simulink model "motor"  (Simulink 8.6)
settings: Solver=FixedStepDiscrete  StartTime=0.0  StopTime=inf  FixedStep=0.002  RelTol=1e-3
PostLoadFcn:
  | ,try, rti_mdl_postloadfcn(bdroot, 'UpdateModel', 160, 'rti1104'); catch, disp(lasterr); end,
undefined symbols (not defined in the file): DiscIntNeverNeededParam
(part 3 of 3)

== stateflow chart Chart ==
  state Ready
    en:
    Cur_Limit=2200;%电流报警阈值
    Cur_GZ_Limit=2450;%电流故障阈值
    Temp_Up_Limit=2130;%温度上限阈值80°C
    Temp_Down_Limit=80;%温度下限阈值-45°C
    Open_Result=2;%开机结果失败
    Ini_Result=0;%初始化结果失败
    QDQ_BJ=1;%默认驱动器正常，1正常，2报警，3故障
    In_State=0;%状态标识，1表示初始化状态，2开机状态，3关机状态
    QDQ_XH=0;%QDQ_XH引脚状态，低
    QDQ_HY=1;%QDQ_HY引脚状态，高
    Motor_En=1;%电机使能引脚置高
    DCZD=1;%电磁制动引脚拉高，关电制动，低有效
    KG_clc=0;
    Alarm_Cunt=1;%实现程序中主动上报只执行发送一次
    Flag_Up_limit=1;%上限位标识，1正常，0报警
    Flag_Down_limit=1;%下限位标识，1正常，0报警
    Flag_Cur=1;%电流报警
    Flag_Temp_Up=1;%温度过高标识
    Flag_GXDY_Error=1;%惯性单元数据异常标识
    Flag_Enc_Error=1;%编码器标识，1正常，0故障
    Flag_Motor_Error=1;%电机正反转标识，1正常，0故障
    Flag_GZ_Cur=1;%电流过高故障
    Flag_Down_GZ_limit= 1;%下限位开关故障标识，1正常，0故障
    Flag_Up_GZ_limit= 1;%上限位开关故障标识，1正常，0故障
    Flag_Temp_Down=1;%温度过低标识，1正常，0故障
    Flag_GXDY_IT=1;%惯性单元通讯中断标识
    PWM_Value_Up= uint16(3300);%电机初始化上行PWM值
    PWM_Value_Down= uint16(1700);%电机初始化下行PWM值
    PWM_Value_Mid= uint16(2500);%PWM中指
    Encode_Sp_Max=3000;%换算编码器测速最大值
    Encode_Sp_Min= uint32(2);%编码器测速最小值
    Encode_Pos1=int32(-1161718);%下滑纵摇XHZY下机械限位位置
    Encode_Pos2=int32(-1155272);%下滑横摇XHHY下机械限位位置
    Encode_Pos3=int32(-1163716);%横摇灯杆XYDG下机械限位位置
    Encode_Pos_Zero=1000;%零点检测，回到零点时的范围
    Encode_Pos_Min=uint32(1400);%最小行程，检测电机是否正常运转
    JD_Max=uint32(20000);%角度变化最大值,
    Ts=double(0.002);%采样时间
  state Ready_Run
    state Current_check [parallel]
      settings: executionOrder=1
      state p1
        entry: cur_i=uint16(0);%计数器置零
        Flag_Cur=uint8(1);%电流正常
      state p4
        en:cur_i= uint16(1);
        du:cur_i = cur_i + 1;
      state p3
        %0代表正常，1代表错误
        entry: cur_i= uint16(0);
        Flag_Cur=uint8(0);%电流过流
        Flag_GZ_Cur=1;%电流未故障
      state p2
        en:cur_i=uint16(1);
        du:cur_i = cur_i + 1;
      state p5
        en:cur_i=uint16(1);
        du:cur_i = cur_i + 1;
      state p7
        en:cur_i= uint16(1);
        du:cur_i = cur_i + 1;
      state p6
        entry:%Motor_En=1;%电机失能
        Flag_GZ_Cur=uint8(0);%电流过流
      (default) -> Ready_Run.Current_check.p1
      Ready_Run.Current_check.p4 -> Ready_Run.Current_check.p1 [order 2] : [cur_i>=uint16(2/Ts)]
      Ready_Run.Current_check.p1 -> Ready_Run.Current_check.p2 : [Cur_In>=Cur_Limit]
      Ready_Run.Current_check.p2 -> Ready_Run.Current_check.p1 [order 1] : [Cur_In<Cur_Limit]
      Ready_Run.Current_check.p4 -> Ready_Run.Current_check.p3 [order 1] : [Cur_In>=Cur_Limit]
      Ready_Run.Current_check.p3 -> Ready_Run.Current_check.p4 [order 1] : [Cur_In<Cur_Limit]
      Ready_Run.Current_check.p7 -> Ready_Run.Current_check.p3 [order 2] : [cur_i>=uint16(2/Ts)]
      Ready_Run.Current_check.p2 -> Ready_Run.Current_check.p3 [order 2] : [cur_i>=uint16(2/Ts)]%2S
      Ready_Run.Current_check.p3 -> Ready_Run.Current_check.p5 [order 2] : [Cur_In>=Cur_GZ_Limit]
      Ready_Run.Current_check.p5 -> Ready_Run.Current_check.p3 [order 2] : [Cur_In<Cur_GZ_Limit]
      Ready_Run.Current_check.p5 -> Ready_Run.Current_check.p6 [order 1] : [cur_i>=uint16(2/Ts)]%2S
      Ready_Run.Current_check.p6 -> Ready_Run.Current_check.p7 : [Cur_In<Cur_GZ_Limit]
      Ready_Run.Current_check.p7 -> Ready_Run.Current_check.p6 [order 1] : [Cur_In>=Cur_GZ_Limit]
    state M_Run [parallel]
      entry:Encode_Pos0=Encode_Sp+Encode_Pos0;
      during:Encode_Pos0=Encode_Sp+Encode_Pos0;
      Encode_Pos=Encode_Pos0-Encode_Pos_Zero_Average;
      settings: executionOrder=3
      state Initialize
        entry:Ini_Result=uint8(0);%初始化失败
        In_State=1;
        state Parameters_Reset
          entry:
          Motor_En=0;%开电机
          Encode_Pos0= int32(0);%位置初始值
          chu_jd=0;
          KG=1;
        state hy
          state P5
            en:PWMOUT=PWM_Value_Up;
            du:PWMOUT=PWM_Value_Up;%电机上行
            on after(4/Ts,tick):Flag_Down_GZ_limit=0;%下限位开关故障
            %Motor_En=1;
            %PWMOUT=PWM_Value_Mid;
            %4S之后停机
          state P3
            en:PWMOUT=PWM_Value_Down;
            du:PWMOUT=PWM_Value_Down;%电机下行*/
            on after(4/Ts,tick):Flag_Up_GZ_limit= uint8(0);%上限位开关故障*/
            %Motor_En=1;
            %电机失能，关
            %PWMOUT=PWM_Value_Mid;
            %4S之后停机*/
          state P4
            en:chu_jd=chu_jd-0.01;
            [PWMOUT,JD_Error,JD_Out] = Motor_HYDG(JD_In,Encode_Pos0,System_Order,Encode_Sp);
            du:chu_jd=chu_jd-0.01;%电机下行
            [PWMOUT,JD_Error,JD_Out] = Motor_HYDG(JD_In,Encode_Pos0,System_Order,Encode_Sp);
            %电机触碰到机械限位
          state P8
            en:Flag_Motor_Error=0;%电机故障，不能正转
            %Motor_En=1;
            %电机失能，关
          state P1
            en:KG_JD=uint8(0);KG_clc=0;
            du:chu_jd=chu_jd+0.01;%电机上行
            [PWMOUT,JD_Error,JD_Out] = Motor_HYDG(JD_In,Encode_Pos0,System_Order,Encode_Sp);
          state p11
            en:Encode_Pos0=Encode_Pos1;
            chu_jd=(-20);
            du:chu_jd=chu_jd+0.01;%电机上行回零点
            [PWMOUT,JD_Error,JD_Out] = Motor_HYDG(JD_In,Encode_Pos,System_Order,Encode_Sp);
          state P2
            en:chu_jd=chu_jd-0.01;
            [PWMOUT,JD_Error,JD_Out] = Motor_HYDG(JD_In,Encode_Pos0,System_Order,Encode_Sp);
            du:chu_jd=chu_jd-0.01;%电机下行
            [PWMOUT,JD_Error,JD_Out] = Motor_HYDG(JD_In,Encode_Pos0,System_Order,Encode_Sp);
          state P10
            en:chu_jd=chu_jd-0.01;
            [PWMOUT,JD_Error,JD_Out] = Motor_HYDG(JD_In,Encode_Pos0,System_Order,Encode_Sp);
            du:chu_jd=chu_jd-0.01;%电机下行
            [PWMOUT,JD_Error,JD_Out] = Motor_HYDG(JD_In,Encode_Pos0,System_Order,Encode_Sp);
            %电机触碰到机械限位
          state P9
            en:Flag_Motor_Error=0;%电机故障，不能反转
            %Motor_En=1;
            %电机失能，关
          state p12
            en:Motor_En=1;%关电机
            PWMOUT=PWM_Value_Mid;
          (default) -> Ready_Run.M_Run.Initialize.hy.P1
          Ready_Run.M_Run.Initialize.hy.P1 -> (junction 362) [order 1] : [after(2/Ts,tick)]
              | %等待3S
          (junction 362) -> Ready_Run.M_Run.Initialize.hy.P8 [order 1] : [Encode_Pos0<=293092]%293092为2.5度
          (junction 362) -> Ready_Run.M_Run.Initialize.hy.P3 [order 2] : [abs(Encode_Sp)<=Encode_Sp_Min]
              | % 判断电机是否到达上机械限位
              | %故障（卡死）
              | %编码器故障
          Ready_Run.M_Run.Initialize.hy.P1 -> Ready_Run.M_Run.Initialize.hy.P2 [order 2] : [Up_Limit==0]
              | %上限位开关低电平有效
          (junction 363) -> Ready_Run.M_Run.Initialize.hy.P5 [order 2] : [abs(Encode_Sp)<=Encode_Sp_Min]
              | % 判断电机是否到达下机械限位
              | %故障（卡死）
          (junction 363) -> Ready_Run.M_Run.Initialize.hy.P9 [order 1] : [Encode_Pos_kj>=Encode_sxwPos_Motor]
          Ready_Run.M_Run.Initialize.hy.P2 -> (junction 363) [order 1] : [after(2/Ts,tick)]%等待5S
          Ready_Run.M_Run.Initialize.hy.P2 -> Ready_Run.M_Run.Initialize.hy.P4 [order 2] : [Down_Limit==0]
              | %下限位开关低电平有效
          Ready_Run.M_Run.Initialize.hy.P4 -> Ready_Run.M_Run.Initialize.hy.P10 : [abs(Encode_Sp)<=Encode_Sp_Min]
              | % 判断电机是否到达下机械限位
          Ready_Run.M_Run.Initialize.hy.P10 -> Ready_Run.M_Run.Initialize.hy.p11 : [after(0.5/Ts,tick)]
          Ready_Run.M_Run.Initialize.hy.p11 -> Ready_Run.M_Run.Initialize.hy.p12 : [abs(chu_jd)<=0.02]
        state xhhy
          state P1
            en:KG_JD=uint8(0);KG_En=uint8(1);KG_clc=~KG_clc;
            chu_jd=chu_jd+0.01;%电机上行
            [PWMOUT,JD_Out,JD_Error] = Motor_XHHY(JD_In,Encode_Pos0,Encode_Sp,System_Order,SGWY_In);
            during:chu_jd=chu_jd+0.01;%电机上行
            [PWMOUT,JD_Out,JD_Error] = Motor_XHHY(JD_In,Encode_Pos0,Encode_Sp,System_Order,SGWY_In);
          state P10
            en:chu_jd=chu_jd+0.01;%电机上行
            [PWMOUT,JD_Out,JD_Error] = Motor_XHHY(JD_In,Encode_Pos0,Encode_Sp,System_Order,SGWY_In);
            during:chu_jd=chu_jd+0.01;%电机上行
            [PWMOUT,JD_Out,JD_Error] = Motor_XHHY(JD_In,Encode_Pos0,Encode_Sp,System_Order,SGWY_In);
            %电机触碰到机械上限位
          state P8
            en:Flag_Motor_Error=0;%电机故障，不能正转
            %Motor_En=1;
            %电机失能，关
          state P5
            en:PWMOUT=PWM_Value_Up;
            du:PWMOUT=PWM_Value_Up;%电机上行
            on after(4/Ts,tick):Flag_Down_GZ_limit=0;%下限位开关故障
            %Motor_En=1;
            %PWMOUT=PWM_Value_Mid;
            %4S之后停机
          state P11
            en:chu_jd=chu_jd-0.01;%电机下行
            [PWMOUT,JD_Out,JD_Error] = Motor_XHHY(JD_In,Encode_Pos0,Encode_Sp,System_Order,SGWY_In);
            du:chu_jd=chu_jd-0.01;%电机下行
            [PWMOUT,JD_Out,JD_Error] = Motor_XHHY(JD_In,Encode_Pos0,Encode_Sp,System_Order,SGWY_In);
            %电机触碰到机械限位
          state P4
            en:chu_jd=chu_jd-0.01;%电机下行
            [PWMOUT,JD_Out,JD_Error] = Motor_XHHY(JD_In,Encode_Pos0,Encode_Sp,System_Order,SGWY_In);
            du:chu_jd=chu_jd-0.01;%电机下行
            [PWMOUT,JD_Out,JD_Error] = Motor_XHHY(JD_In,Encode_Pos0,Encode_Sp,System_Order,SGWY_In);
            %电机触碰到机械限位
          state p10
            en:Encode_Pos0=Encode_Pos2;
            chu_jd=(-20);
            du:chu_jd=chu_jd+0.01;%电机上行回零点
            [PWMOUT,JD_Out,JD_Error] = Motor_XHHY(JD_In,Encode_Pos,Encode_Sp,System_Order,SGWY_In);
          state P2
            en:chu_jd=chu_jd-0.01;%电机下行
            [PWMOUT,JD_Out,JD_Error] = Motor_XHHY(JD_In,Encode_Pos0,Encode_Sp,System_Order,SGWY_In);
            du:chu_jd=chu_jd-0.01;%电机下行
            [PWMOUT,JD_Out,JD_Error] = Motor_XHHY(JD_In,Encode_Pos0,Encode_Sp,System_Order,SGWY_In);
          state P9
            en:Flag_Motor_Error=0;%电机故障，不能反转
            %Motor_En=1;
            %电机失能，关
          state p11
            en:Motor_En=1;%关电机
            PWMOUT=PWM_Value_Mid;
          state P3
            en:PWMOUT=PWM_Value_Down;
            du:PWMOUT=PWM_Value_Down;%电机下行*/
            on after(4/Ts,tick):Flag_Up_GZ_limit= uint8(0);%上限位开关故障*/
            %Motor_En=1;
            %电机失能，关
            %PWMOUT=PWM_Value_Mid;
            %4S之后停机*/
          (default) -> Ready_Run.M_Run.Initialize.xhhy.P1
          Ready_Run.M_Run.Initialize.xhhy.P1 -> (junction 377) [order 2] : [after(2/Ts,tick)]
              | %等待3S
          (junction 377) -> Ready_Run.M_Run.Initialize.xhhy.P8 [order 1] : [Encode_Pos0<=293092]%293092为2.5度
          (junction 377) -> Ready_Run.M_Run.Initialize.xhhy.P3 [order 2] : [abs(Encode_Sp)<=Encode_Sp_Min]
              | % 判断电机是否到达上机械限位
              | %故障（卡死）
              | %编码器故障
          Ready_Run.M_Run.Initialize.xhhy.P1 -> Ready_Run.M_Run.Initialize.xhhy.P10 [order 1] : [Up_Limit==0]
              | %上限位开关低电平有效
          Ready_Run.M_Run.Initialize.xhhy.P10 -> Ready_Run.M_Run.Initialize.xhhy.P2 : [abs(Encode_Sp)<=Encode_Sp_Min]
              | % 判断电机是否到达上机械限位
          Ready_Run.M_Run.Initialize.xhhy.P2 -> (junction 378) [order 1] : [after(2/Ts,tick)]%等待5S
          (junction 378) -> Ready_Run.M_Run.Initialize.xhhy.P5 [order 2] : [abs(Encode_Sp)<=Encode_Sp_Min]
              | % 判断电机是否到达下机械限位
              | %故障（卡死）
          (junction 378) -> Ready_Run.M_Run.Initialize.xhhy.P9 [order 1] : [Encode_Pos_kj>=Encode_sxwPos_Motor]
          Ready_Run.M_Run.Initialize.xhhy.P2 -> Ready_Run.M_Run.Initialize.xhhy.P4 [order 2] : [Down_Limit==0]
              | %下限位开关低电平有效
          Ready_Run.M_Run.Initialize.xhhy.P4 -> P11 : [abs(Encode_Sp)<=Encode_Sp_Min]
              | % 判断电机是否到达下机械限位
          P11 -> p10 : [after(0.5/Ts,tick)]
          p10 -> Ready_Run.M_Run.Initialize.xhhy.p11 : [abs(chu_jd)<=0.02]
        state Check_Reset
          entry:
          Ini_Result=Init_Result_Check(Flag_Cur,Flag_Temp_Up,Flag_Temp_Down);
          DCZD=1;%开启制动
          during:
          Ini_Result=Init_Result_Check(Flag_Cur,Flag_Temp_Up,Flag_Temp_Down);
        state Parameters_Reset0
          entry:
          DCZD=0;%解除制动
        state xhzy
          state P9
            en:Flag_Motor_Error=0;%电机故障，不能反转
            %Motor_En=1;
            %电机失能，关
          state P8
            en:Flag_Motor_Error=0;%电机故障，不能正转
            %Motor_En=1;
            %电机失能，关
          state P10
            en:chu_jd=chu_jd-0.01;%电机下行;
            [PWMOUT,JD_Out,JD_Error] = Motor_XHHY(JD_In,Encode_Pos0,Encode_Sp,System_Order,SGWY_In);
            du:chu_jd=chu_jd-0.01;%电机下行;
            [PWMOUT,JD_Out,JD_Error] = Motor_XHHY(JD_In,Encode_Pos0,Encode_Sp,System_Order,SGWY_In);
            %电机下行
            %电机触碰到机械限位
          state P5
            en:PWMOUT=PWM_Value_Up;
            du:PWMOUT=PWM_Value_Up;%电机上行
            on after(4/Ts,tick):Flag_Down_GZ_limit=0;%下限位开关故障
            %Motor_En=1;
            %PWMOUT=PWM_Value_Mid;
            %4S之后停机
          state P1
            en:KG_JD=uint8(0);KG_En=uint8(1);KG_clc=0;
            chu_jd=chu_jd+0.01;%电机上行
            [PWMOUT,JD_Out,JD_Error] = Motor_XHHY(JD_In,Encode_Pos0,Encode_Sp,System_Order,SGWY_In);
            during:chu_jd=chu_jd+0.01;%电机上行;
            [PWMOUT,JD_Out,JD_Error] = Motor_XHHY(JD_In,Encode_Pos0,Encode_Sp,System_Order,SGWY_In);
            %电机上行
          state P2
            en:chu_jd=chu_jd-0.01;%电机下行;
            [PWMOUT,JD_Out,JD_Error] = Motor_XHHY(JD_In,Encode_Pos0,Encode_Sp,System_Order,SGWY_In);
            du:chu_jd=chu_jd-0.01;%电机下行;
            [PWMOUT,JD_Out,JD_Error] = Motor_XHHY(JD_In,Encode_Pos0,Encode_Sp,System_Order,SGWY_In);
            %电机下行
          state P4
            en:chu_jd=chu_jd-0.01;%电机下行;
            [PWMOUT,JD_Out,JD_Error] = Motor_XHHY(JD_In,Encode_Pos0,Encode_Sp,System_Order,SGWY_In);
            du:chu_jd=chu_jd-0.01;%电机下行;
            [PWMOUT,JD_Out,JD_Error] = Motor_XHHY(JD_In,Encode_Pos0,Encode_Sp,System_Order,SGWY_In);
            %电机下行
            %电机触碰到机械限位
          state p12
            en:Motor_En=1;%关电机
            PWMOUT=PWM_Value_Mid;
          state p11
            en:Encode_Pos0=Encode_Pos1;
            chu_jd=(-20);
            du:chu_jd=chu_jd+0.01;%电机上行回零点
            [PWMOUT,JD_Out,JD_Error] = Motor_XHHY(JD_In,Encode_Pos,Encode_Sp,System_Order,SGWY_In);
          state P3
            en:PWMOUT=PWM_Value_Down;
            du:PWMOUT=PWM_Value_Down;%电机下行*/
            on after(4/Ts,tick):Flag_Up_GZ_limit= uint8(0);%上限位开关故障*/
            %Motor_En=1;
            %电机失能，关
            %PWMOUT=PWM_Value_Mid;
            %4S之后停机*/
          (default) -> Ready_Run.M_Run.Initialize.xhzy.P1
          Ready_Run.M_Run.Initialize.xhzy.P1 -> (junction 439) [order 1] : [after(2/Ts,tick)]
              | %等待3S
          (junction 439) -> Ready_Run.M_Run.Initialize.xhzy.P8 [order 1] : [Encode_Pos0<=293092]%293092为2.5度
          (junction 439) -> Ready_Run.M_Run.Initialize.xhzy.P3 [order 2] : [abs(Encode_Sp)<=Encode_Sp_Min]
              | % 判断电机是否到达上机械限位
              | %故障（卡死）
              | %编码器故障
          Ready_Run.M_Run.Initialize.xhzy.P1 -> Ready_Run.M_Run.Initialize.xhzy.P2 [order 2] : [Up_Limit==0]
              | %上限位开关低电平有效
          (junction 440) -> Ready_Run.M_Run.Initialize.xhzy.P5 [order 2] : [abs(Encode_Sp)<=Encode_Sp_Min]
              | % 判断电机是否到达下机械限位
              | %故障（卡死）
          (junction 440) -> Ready_Run.M_Run.Initialize.xhzy.P9 [order 1] : [Encode_Pos_kj>=Encode_sxwPos_Motor]
          Ready_Run.M_Run.Initialize.xhzy.P2 -> (junction 440) [order 1] : [after(2/Ts,tick)]%等待5S
          Ready_Run.M_Run.Initialize.xhzy.P2 -> Ready_Run.M_Run.Initialize.xhzy.P4 [order 2] : [Down_Limit==0]
              | %下限位开关低电平有效
          Ready_Run.M_Run.Initialize.xhzy.P4 -> Ready_Run.M_Run.Initialize.xhzy.P10 : [abs(Encode_Sp)<=Encode_Sp_Min]
              | % 判断电机是否到达下机械限位
          Ready_Run.M_Run.Initialize.xhzy.P10 -> Ready_Run.M_Run.Initialize.xhzy.p11 : [after(0.5/Ts,tick)]
          Ready_Run.M_Run.Initialize.xhzy.p11 -> Ready_Run.M_Run.Initialize.xhzy.p12 : [abs(chu_jd)<=0.02]
        (default) -> Parameters_Reset0
        (junction 283) -> xhhy [order 2] : [Motor_Num==3]
        Parameters_Reset0 -> Parameters_Reset : [after(0.2/Ts,tick)]
        Parameters_Reset -> (junction 283)
        (junction 283) -> hy [order 3] : [Motor_Num==2]
        (junction 283) -> xhzy [order 1] : [Motor_Num==1]
        (junction 284) -> Check_Reset
        Ready_Run.M_Run.Initialize.xhhy.p11 -> (junction 284) : [after(0.2/Ts,tick)]
        Ready_Run.M_Run.Initialize.hy.p12 -> (junction 284) : [after(0.2/Ts,tick)]
        Ready_Run.M_Run.Initialize.xhzy.p12 -> (junction 284) : [after(0.2/Ts,tick)]
      state Normal_Mode
        %正常模式
        entry:
        DCZD=0;%开电磁制动，低有效
        Open_Result=2;%开机状态位失败
        PWMOUT=PWM_Value_Mid;
        state p1
          state Enc_GZ [parallel]
            entry:Enc_i=0;
            settings: executionOrder=2
            state Enc2 [parallel]
              settings: executionOrder=2
              state p2
              state p5
                entry:Flag_Enc_Error=1;
                Enc_i=0;
              state p3
                entry:Flag_Enc_Error=0;
                during:Flag_Enc_Error=0;
                %Motor_En=1;
              (default) -> Ready_Run.M_Run.Normal_Mode.p1.Enc_GZ.Enc2.p2
              Ready_Run.M_Run.Normal_Mode.p1.Enc_GZ.Enc2.p5 -> Ready_Run.M_Run.Normal_Mode.p1.Enc_GZ.Enc2.p2
              Ready_Run.M_Run.Normal_Mode.p1.Enc_GZ.Enc2.p2 -> (junction 302) : [every(5/Ts,tick)]%5秒钟
              (junction 302) -> Ready_Run.M_Run.Normal_Mode.p1.Enc_GZ.Enc2.p5 [order 2] : [Enc_i<100]
              (junction 302) -> Ready_Run.M_Run.Normal_Mode.p1.Enc_GZ.Enc2.p3 [order 1] : [Enc_i>=100]
            state Enc1 [parallel]
              settings: executionOrder=1
              state p1
                entry:Flag_Enc_Error=1;
              state p4
                entry:Enc_i=Enc_i+1;
                during:Enc_i=Enc_i+1;
              (default) -> Ready_Run.M_Run.Normal_Mode.p1.Enc_GZ.Enc1.p1
              Ready_Run.M_Run.Normal_Mode.p1.Enc_GZ.Enc1.p1 -> Ready_Run.M_Run.Normal_Mode.p1.Enc_GZ.Enc1.p4 : [abs(Encode_Sp)>Encode_Sp_Max]
              Ready_Run.M_Run.Normal_Mode.p1.Enc_GZ.Enc1.p4 -> Ready_Run.M_Run.Normal_Mode.p1.Enc_GZ.Enc1.p1 : [abs(Encode_Sp)<=Encode_Sp_Max]
          state RUN [parallel]
            settings: executionOrder=1
            state GXDY_SJ_BJ [parallel]
              during:JD_Vary = COM_Error(JD_In);
              settings: executionOrder=2
              state p2
                en:can1_i=uint16(1);
                du:can1_i = can1_i + 1;
              state p4
                en:can1_i= uint16(1);
                du:can1_i = can1_i + 1;
              note: CAN收到数据，但是数据不对,
                  | 大于速度最大值
              state p3
                %0代表正常，1代表错误
                entry: can1_i= uint16(0);
                %Motor_En=uint8(1);%电机失能
                Flag_GXDY_Error=uint8(0);
                %惯性单元通讯故障
              state Defult
              state p1
                entry: can1_i=uint16(0);%计数器置零
                du:Flag_GXDY_Error=uint8(1);
                %惯性单元正常
              (default) -> Ready_Run.M_Run.Normal_Mode.p1.RUN.GXDY_SJ_BJ.Defult
              Ready_Run.M_Run.Normal_Mode.p1.RUN.GXDY_SJ_BJ.Defult -> Ready_Run.M_Run.Normal_Mode.p1.RUN.GXDY_SJ_BJ.p1 : [Open_Result==1&&GXDY_State==0]
                  | %开机成功且惯性单元打开
              Ready_Run.M_Run.Normal_Mode.p1.RUN.GXDY_SJ_BJ.p4 -> Ready_Run.M_Run.Normal_Mode.p1.RUN.GXDY_SJ_BJ.p1 [order 2] : [can1_i>=2/Ts]
              Ready_Run.M_Run.Normal_Mode.p1.RUN.GXDY_SJ_BJ.p4 -> Ready_Run.M_Run.Normal_Mode.p1.RUN.GXDY_SJ_BJ.p3 [order 1] : [JD_Vary>JD_Max]
              Ready_Run.M_Run.Normal_Mode.p1.RUN.GXDY_SJ_BJ.p3 -> Ready_Run.M_Run.Normal_Mode.p1.RUN.GXDY_SJ_BJ.p4 : [JD_Vary<=JD_Max]
              Ready_Run.M_Run.Normal_Mode.p1.RUN.GXDY_SJ_BJ.p1 -> Ready_Run.M_Run.Normal_Mode.p1.RUN.GXDY_SJ_BJ.p2 : [JD_Vary>JD_Max]
                  | %速度大于最大值
              Ready_Run.M_Run.Normal_Mode.p1.RUN.GXDY_SJ_BJ.p2 -> Ready_Run.M_Run.Normal_Mode.p1.RUN.GXDY_SJ_BJ.p1 [order 1] : [JD_Vary<=JD_Max]
              Ready_Run.M_Run.Normal_Mode.p1.RUN.GXDY_SJ_BJ.p2 -> Ready_Run.M_Run.Normal_Mode.p1.RUN.GXDY_SJ_BJ.p3 [order 2] : [can1_i>=2/Ts]%2S
            state GXDY_COM_GZ [parallel]
              settings: executionOrder=1
              state p5
                en:GXDY_i=1;
                du:GXDY_i = GXDY_i + 1;
              state r2
                entry:
                Flag_GXDY_IT=0;%故障
              state p7
                entry:
                GXDY_i=0;%计数器置零
                Flag_GXDY_IT=1;%正常
              state p6
                %1代表正常，0代表错误
                entry:
                Flag_GXDY_IT=0;%故障
                %Motor_En=1;%电机失能
              state Defult
              Ready_Run.M_Run.Normal_Mode.p1.RUN.GXDY_COM_GZ.Defult -> (junction 501) [order 2] : [Open_Result==1]
                  | %开机成功
              (junction 501) -> (junction 502) : after(10/Ts,tick)
              (default) -> Ready_Run.M_Run.Normal_Mode.p1.RUN.GXDY_COM_GZ.Defult
              Ready_Run.M_Run.Normal_Mode.p1.RUN.GXDY_COM_GZ.Defult -> Ready_Run.M_Run.Normal_Mode.p1.RUN.GXDY_COM_GZ.p7 [order 1] : [Open_Result==1&&GXDY_State==0]
                  | %开机成功且惯性单元打开
              (junction 502) -> Ready_Run.M_Run.Normal_Mode.p1.RUN.GXDY_COM_GZ.r2 : [GXDY_State==1]
              Ready_Run.M_Run.Normal_Mode.p1.RUN.GXDY_COM_GZ.p7 -> Ready_Run.M_Run.Normal_Mode.p1.RUN.GXDY_COM_GZ.p5 : [GXDY_IT_In==0]
              Ready_Run.M_Run.Normal_Mode.p1.RUN.GXDY_COM_GZ.p5 -> Ready_Run.M_Run.Normal_Mode.p1.RUN.GXDY_COM_GZ.p7 [order 1] : [GXDY_IT_In==1]
              Ready_Run.M_Run.Normal_Mode.p1.RUN.GXDY_COM_GZ.p5 -> Ready_Run.M_Run.Normal_Mode.p1.RUN.GXDY_COM_GZ.p6 [order 2] : [GXDY_i>=uint16(3/Ts)]%3S
            state Algorithm [parallel]
              settings: executionOrder=4
              state Defualt
                en:chu_jd=0;
                KG=0;
                KG_clc=1;
                Motor_En=0;
              state XHHY
                state Defualt
                  entry:
                  %en:KG_En=uint8(0);KG_JD=uint8(1);KG_YJ=uint8(1);
                  KG_En=uint8(1);KG_JD=uint8(0);KG_clc=~KG_clc;
                  during:[PWMOUT,JD_Out,JD_Error] = Motor_XHHY(JD_In,Encode_Pos,Encode_Sp,System_Order,SGWY_In);
                state XHHY_Run
                  en:KG_En=uint8(0);KG_JD=uint8(1);KG_clc=~KG_clc;
                  %外部接口
                  during:KG_JD=uint8(1);
                  [PWMOUT,JD_Out,JD_Error] = Motor_XHHY(JD_In,Encode_Pos,Encode_Sp,System_Order,SGWY_In);
                state XHHY_Error
                  en:Motor_En=uint8(1);%关电机
                state Sleeping_protect_2
                  entry:
                  DCZD=1;%关电磁制动
                  exit:
                  DCZD=0;%开电磁制动
                state XHHY_Wait
                  en:Open_Result=uint8(1);
                  %开机状态位成功
                  In_State=2;
                  KG_En=uint8(1);KG_clc=~KG_clc;
                  during:[PWMOUT,JD_Out,JD_Error] = Motor_XHHY(JD_In,Encode_Pos,Encode_Sp,System_Order,SGWY_In);
                  %PWMOUT=2500;
                state Sleeping_protect_3
                  entry:
                  Motor_En=0;%开电机
                state Sleeping_protect_1
                  entry:
                  Motor_En=1;%关电机
                  PWMOUT=PWM_Value_Mid;
                (default) -> Ready_Run.M_Run.Normal_Mode.p1.RUN.Algorithm.XHHY.Defualt
                Ready_Run.M_Run.Normal_Mode.p1.RUN.Algorithm.XHHY.Sleeping_protect_1 -> Ready_Run.M_Run.Normal_Mode.p1.RUN.Algorithm.XHHY.Sleeping_protect_2 : [after(0.5/Ts,tick)]
                Ready_Run.M_Run.Normal_Mode.p1.RUN.Algorithm.XHHY.Defualt -> Ready_Run.M_Run.Normal_Mode.p1.RUN.Algorithm.XHHY.XHHY_Wait [order 1] : [abs(Encode_Pos)<=Encode_Pos_Zero]
                Ready_Run.M_Run.Normal_Mode.p1.RUN.Algorithm.XHHY.Defualt -> Ready_Run.M_Run.Normal_Mode.p1.RUN.Algorithm.XHHY.XHHY_Error [order 2] : [after(10/Ts,tick)]
                Ready_Run.M_Run.Normal_Mode.p1.RUN.Algorithm.XHHY.Sleeping_protect_2 -> Ready_Run.M_Run.Normal_Mode.p1.RUN.Algorithm.XHHY.Sleeping_protect_3 : [System_Order==5]
                Ready_Run.M_Run.Normal_Mode.p1.RUN.Algorithm.XHHY.XHHY_Run -> Ready_Run.M_Run.Normal_Mode.p1.RUN.Algorithm.XHHY.Sleeping_protect_1 [order 2] : [System_Order==4]
                Ready_Run.M_Run.Normal_Mode.p1.RUN.Algorithm.XHHY.Sleeping_protect_3 -> Ready_Run.M_Run.Normal_Mode.p1.RUN.Algorithm.XHHY.XHHY_Run : [after(0.5/Ts,tick)]
                Ready_Run.M_Run.Normal_Mode.p1.RUN.Algorithm.XHHY.XHHY_Wait -> Ready_Run.M_Run.Normal_Mode.p1.RUN.Algorithm.XHHY.XHHY_Run : [GXDY_State==0]
                    | %惯性单元拉低
              state HY
                state XHHY_Error
                  en:Motor_En=uint8(1);%关电机
                state Sleeping_protect_2
                  entry:
                  DCZD=1;%关电磁制动
                  exit:
                  DCZD=0;%开电磁制动
                state Defualt1
                  entry:
                  KG_JD=uint8(0);
                  during:[PWMOUT,JD_Error,JD_Out] = Motor_HYDG(JD_In,Encode_Pos,System_Order,Encode_Sp);
                state XHHY_Run
                  en:KG_JD=uint8(1);
                  %外部接口
                  during:%[PWMOUT,JD_Error,JD_Out] = Motor_HYDG1(JD_In,Encode_Pos,System_Order):
                  [PWMOUT,JD_Error,JD_Out] = Motor_HYDG1(JD_In,Encode_Pos,System_Order);
                state XHHY_Wait
                  en:Open_Result=uint8(1);
                  %开机状态位成功
                  In_State=2;
                  during:[PWMOUT,JD_Error,JD_Out] = Motor_HYDG(JD_In,Encode_Pos,System_Order,Encode_Sp);
                  %PWMOUT=2500;
                state Sleeping_protect_3
                  entry:
                  Motor_En=0;%开电机
                state Sleeping_protect_1
                  entry:
                  Motor_En=1;%关电机
                  PWMOUT=PWM_Value_Mid;
                (default) -> Ready_Run.M_Run.Normal_Mode.p1.RUN.Algorithm.HY.Defualt1
                Ready_Run.M_Run.Normal_Mode.p1.RUN.Algorithm.HY.Sleeping_protect_1 -> Ready_Run.M_Run.Normal_Mode.p1.RUN.Algorithm.HY.Sleeping_protect_2 : [after(0.5/Ts,tick)]
                Ready_Run.M_Run.Normal_Mode.p1.RUN.Algorithm.HY.Defualt1 -> Ready_Run.M_Run.Normal_Mode.p1.RUN.Algorithm.HY.XHHY_Wait [order 1] : [abs(Encode_Pos)<=Encode_Pos_Zero]
                Ready_Run.M_Run.Normal_Mode.p1.RUN.Algorithm.HY.Defualt1 -> Ready_Run.M_Run.Normal_Mode.p1.RUN.Algorithm.HY.XHHY_Error [order 2] : [after(10/Ts,tick)]
                Ready_Run.M_Run.Normal_Mode.p1.RUN.Algorithm.HY.Sleeping_protect_2 -> Ready_Run.M_Run.Normal_Mode.p1.RUN.Algorithm.HY.Sleeping_protect_3 : [System_Order==5]
                Ready_Run.M_Run.Normal_Mode.p1.RUN.Algorithm.HY.XHHY_Run -> Ready_Run.M_Run.Normal_Mode.p1.RUN.Algorithm.HY.Sleeping_protect_1 [order 2] : [System_Order==4]
                Ready_Run.M_Run.Normal_Mode.p1.RUN.Algorithm.HY.Sleeping_protect_3 -> Ready_Run.M_Run.Normal_Mode.p1.RUN.Algorithm.HY.XHHY_Run : [after(0.5/Ts,tick)]
                Ready_Run.M_Run.Normal_Mode.p1.RUN.Algorithm.HY.XHHY_Wait -> (junction 523) : after(5,tick)
                (junction 523) -> Ready_Run.M_Run.Normal_Mode.p1.RUN.Algorithm.HY.XHHY_Run : [GXDY_State==0]
                    | %惯性单元拉低
              state XHZY
                state XHZY_Run
                  en:KG_En=uint8(0);KG_JD=uint8(1);KG_YJ=uint8(1);KG_clc=~KG_clc;
                  %KG_YJ=uint8(1);%接入外部接口
                  during:[PWMOUT,JD_Out,JD_Error,SGWY_Out] = Motor_XHZY(JD_In,Encode_Pos,YJ_In,Encode_Sp,System_Order);
                state Defualt
                  entry:
                  %en:KG_En=uint8(0);KG_JD=uint8(1);KG_YJ=uint8(1);
                  KG_En=uint8(1);KG_JD=uint8(0);KG_YJ=uint8(0);KG_clc=~KG_clc;
                  during:[PWMOUT,JD_Out,JD_Error,SGWY_Out] = Motor_XHZY(JD_In,Encode_Pos,YJ_In,Encode_Sp,System_Order);
                state XHZY_Error
                  en:Motor_En=1;%电机失能
                state XHZY_Wait
                  en:Open_Result=1;
                  %开机状态位成功
                  In_State=2;
                  KG_En=uint8(1);KG_clc=~KG_clc;
                  during:[PWMOUT,JD_Out,JD_Error,SGWY_Out] = Motor_XHZY(JD_In,Encode_Pos,YJ_In,Encode_Sp,System_Order);
                  %PWMOUT=2500;
                state Sleeping_protect_3
                  entry:
                  Motor_En=0;%开电机
                state Sleeping_protect_1
                  entry:
                  Motor_En=1;%关电机
                  PWMOUT=PWM_Value_Mid;
                state Sleeping_protect_2
                  entry:
                  DCZD=1;%关电磁制动
                  exit:
                  DCZD=0;%开电磁制动
                (default) -> Ready_Run.M_Run.Normal_Mode.p1.RUN.Algorithm.XHZY.Defualt
                Ready_Run.M_Run.Normal_Mode.p1.RUN.Algorithm.XHZY.Defualt -> Ready_Run.M_Run.Normal_Mode.p1.RUN.Algorithm.XHZY.XHZY_Wait [order 2] : [abs(Encode_Pos)<=Encode_Pos_Zero]
                Ready_Run.M_Run.Normal_Mode.p1.RUN.Algorithm.XHZY.Defualt -> Ready_Run.M_Run.Normal_Mode.p1.RUN.Algorithm.XHZY.XHZY_Error [order 1] : [after(15/Ts,tick)]%等待15s
                Ready_Run.M_Run.Normal_Mode.p1.RUN.Algorithm.XHZY.Sleeping_protect_1 -> Ready_Run.M_Run.Normal_Mode.p1.RUN.Algorithm.XHZY.Sleeping_protect_2 : [after(0.5/Ts,tick)]
                Ready_Run.M_Run.Normal_Mode.p1.RUN.Algorithm.XHZY.Sleeping_protect_2 -> Ready_Run.M_Run.Normal_Mode.p1.RUN.Algorithm.XHZY.Sleeping_protect_3 : [System_Order==5]
                Ready_Run.M_Run.Normal_Mode.p1.RUN.Algorithm.XHZY.XHZY_Run -> Ready_Run.M_Run.Normal_Mode.p1.RUN.Algorithm.XHZY.Sleeping_protect_1 [order 2] : [System_Order==4]
                Ready_Run.M_Run.Normal_Mode.p1.RUN.Algorithm.XHZY.XHZY_Wait -> (junction 534) : after(5,tick)
                Ready_Run.M_Run.Normal_Mode.p1.RUN.Algorithm.XHZY.Sleeping_protect_3 -> Ready_Run.M_Run.Normal_Mode.p1.RUN.Algorithm.XHZY.XHZY_Run : [after(0.5/Ts,tick)]
                (junction 534) -> Ready_Run.M_Run.Normal_Mode.p1.RUN.Algorithm.XHZY.XHZY_Run : [GXDY_State==0]
                    | %惯性单元拉低
              (default) -> Ready_Run.M_Run.Normal_Mode.p1.RUN.Algorithm.Defualt
              Ready_Run.M_Run.Normal_Mode.p1.RUN.Algorithm.Defualt -> Ready_Run.M_Run.Normal_Mode.p1.RUN.Algorithm.XHHY [order 1] : [Motor_Num==3]
              Ready_Run.M_Run.Normal_Mode.p1.RUN.Algorithm.Defualt -> Ready_Run.M_Run.Normal_Mode.p1.RUN.Algorithm.HY [order 2] : [Motor_Num==2]
              Ready_Run.M_Run.Normal_Mode.p1.RUN.Algorithm.Defualt -> Ready_Run.M_Run.Normal_Mode.p1.RUN.Algorithm.XHZY [order 3] : [Motor_Num==1]
              Ready_Run.M_Run.Normal_Mode.p1.RUN.Algorithm.XHZY.XHZY_Run -> (junction 511) [order 1] : [System_Order==3]
              Ready_Run.M_Run.Normal_Mode.p1.RUN.Algorithm.XHHY.XHHY_Run -> (junction 511) [order 1] : [System_Order==3]
              Ready_Run.M_Run.Normal_Mode.p1.RUN.Algorithm.HY.XHHY_Run -> (junction 511) [order 1] : [System_Order==3]
            state Limit_Check [parallel]
              settings: executionOrder=3
              state p2
                entry:Flag_Up_limit=0;
              state p3
                entry: Flag_Down_limit=0;
              state defult
              state p1
                entry:
                Flag_Down_limit=1;
                Flag_Up_limit=1;
                Flag_Up_GZ_limit=1;
                Flag_Down_GZ_limit=1;
              (default) -> Ready_Run.M_Run.Normal_Mode.p1.RUN.Limit_Check.defult
              Ready_Run.M_Run.Normal_Mode.p1.RUN.Limit_Check.defult -> Ready_Run.M_Run.Normal_Mode.p1.RUN.Limit_Check.p1 : [after(1/Ts,tick)]
              Ready_Run.M_Run.Normal_Mode.p1.RUN.Limit_Check.p1 -> Ready_Run.M_Run.Normal_Mode.p1.RUN.Limit_Check.p2 [order 1] : [Up_Limit==0]
              Ready_Run.M_Run.Normal_Mode.p1.RUN.Limit_Check.p2 -> Ready_Run.M_Run.Normal_Mode.p1.RUN.Limit_Check.p1 : [Up_Limit==1]
              Ready_Run.M_Run.Normal_Mode.p1.RUN.Limit_Check.p1 -> Ready_Run.M_Run.Normal_Mode.p1.RUN.Limit_Check.p3 [order 2] : [Down_Limit==0]
              Ready_Run.M_Run.Normal_Mode.p1.RUN.Limit_Check.p3 -> Ready_Run.M_Run.Normal_Mode.p1.RUN.Limit_Check.p1 : [Down_Limit==1]
            (default) -> Ready_Run.M_Run.Normal_Mode.p1.RUN.Algorithm
        state defult
        (default) -> Ready_Run.M_Run.Normal_Mode.defult
        Ready_Run.M_Run.Normal_Mode.defult -> Ready_Run.M_Run.Normal_Mode.p1 : [after(1/Ts,tick)]
      state Test_Mode
        %调试模式
        state Calibration
          %标定模式
          entry:
          DCZD=0;%解除制动
          Motor_En=1;%电机失能
          chu_jd=0;
          KG=1;
        state Limit_Up_Test
          %测试电子上限位
          state XHHY
            %下滑横摇电子上限位测试
            state Int6
              entry:
              DCZD=1;%开启制动
            state Int3
              entry:
              chu_jd=chu_jd-0.01;
              [PWMOUT,JD_Out,JD_Error] = Motor_XHHY(JD_In,Encode_Pos,Encode_Sp,System_Order,SGWY_In);
              during:
              chu_jd=chu_jd-0.01;
              [PWMOUT,JD_Out,JD_Error] = Motor_XHHY(JD_In,Encode_Pos,Encode_Sp,System_Order,SGWY_In);
            state Int
              en:
              Angle_Calculation=Angle_Calculation_XH(Encode_Pos);
              chu_jd=Angle_Calculation;
              DCZD=0;%解除制动
              Motor_En=0;%电机使能
              PWMOUT=PWM_Value_Mid;
              KG=1;
              KG_JD=uint8(0);
              KG_En=uint8(1);
              KG_clc=~KG_clc;
            state Int5
              entry:
              Motor_En=1;%电机失能
              PWMOUT=PWM_Value_Mid;
            state Int4
              entry:
              chu_jd=0;
              [PWMOUT,JD_Out,JD_Error] = Motor_XHHY(JD_In,Encode_Pos,Encode_Sp,System_Order,SGWY_In);
              during:
              [PWMOUT,JD_Out,JD_Error] = Motor_XHHY(JD_In,Encode_Pos,Encode_Sp,System_Order,SGWY_In);
            state Int1
              entry:
              chu_jd=chu_jd+0.002;
              [PWMOUT,JD_Out,JD_Error] = Motor_XHHY(JD_In,Encode_Pos,Encode_Sp,System_Order,SGWY_In);
              during:
              chu_jd=chu_jd+0.002;
              [PWMOUT,JD_Out,JD_Error] = Motor_XHHY(JD_In,Encode_Pos,Encode_Sp,System_Order,SGWY_In);
            state Int2
              entry:
              chu_jd=chu_jd+0.002;
              [PWMOUT,JD_Out,JD_Error] = Motor_XHHY(JD_In,Encode_Pos,Encode_Sp,System_Order,SGWY_In);
              during:
              chu_jd=chu_jd+0.002;
              [PWMOUT,JD_Out,JD_Error] = Motor_XHHY(JD_In,Encode_Pos,Encode_Sp,System_Order,SGWY_In);
            (default) -> Ready_Run.M_Run.Test_Mode.Limit_Up_Test.XHHY.Int
            Ready_Run.M_Run.Test_Mode.Limit_Up_Test.XHHY.Int -> Ready_Run.M_Run.Test_Mode.Limit_Up_Test.XHHY.Int1 : [after(0.5/Ts,tick)]
            Ready_Run.M_Run.Test_Mode.Limit_Up_Test.XHHY.Int1 -> Ready_Run.M_Run.Test_Mode.Limit_Up_Test.XHHY.Int2 : [Up_Limit==0]
                | %上限位开关低电平有效
            Ready_Run.M_Run.Test_Mode.Limit_Up_Test.XHHY.Int2 -> Ready_Run.M_Run.Test_Mode.Limit_Up_Test.XHHY.Int3 : [after(50,tick)]
            Ready_Run.M_Run.Test_Mode.Limit_Up_Test.XHHY.Int3 -> Ready_Run.M_Run.Test_Mode.Limit_Up_Test.XHHY.Int4 : [abs(chu_jd)<0.1]
            Ready_Run.M_Run.Test_Mode.Limit_Up_Test.XHHY.Int5 -> Ready_Run.M_Run.Test_Mode.Limit_Up_Test.XHHY.Int6 : [after(0.5/Ts,tick)]
            Ready_Run.M_Run.Test_Mode.Limit_Up_Test.XHHY.Int4 -> Ready_Run.M_Run.Test_Mode.Limit_Up_Test.XHHY.Int5 : [after(2/Ts,tick)]
          state XHZY
            %下滑纵摇电子上限位测试
            state Int
              en:
              Angle_Calculation=Angle_Calculation_XH(Encode_Pos);
              chu_jd=Angle_Calculation;
              DCZD=0;%解除制动
              Motor_En=0;%电机使能
              PWMOUT=PWM_Value_Mid;
              KG=1;
              KG_JD=uint8(0);
              KG_YJ=uint8(0);
              KG_En=uint8(1);
              KG_clc=~KG_clc;
            state Int1
              entry:
              chu_jd=chu_jd+0.002;
              [PWMOUT,JD_Out,JD_Error,SGWY_Out] = Motor_XHZY(JD_In,Encode_Pos,YJ_In,Encode_Sp,System_Order);
              during:
              chu_jd=chu_jd+0.002;
              [PWMOUT,JD_Out,JD_Error,SGWY_Out] = Motor_XHZY(JD_In,Encode_Pos,YJ_In,Encode_Sp,System_Order);
            state Int2
              entry:
              chu_jd=chu_jd+0.002;
              [PWMOUT,JD_Out,JD_Error,SGWY_Out] = Motor_XHZY(JD_In,Encode_Pos,YJ_In,Encode_Sp,System_Order);
              during:
              chu_jd=chu_jd+0.002;
              [PWMOUT,JD_Out,JD_Error,SGWY_Out] = Motor_XHZY(JD_In,Encode_Pos,YJ_In,Encode_Sp,System_Order);
            state Int3
              entry:
              chu_jd=chu_jd-0.01;
              [PWMOUT,JD_Out,JD_Error,SGWY_Out] = Motor_XHZY(JD_In,Encode_Pos,YJ_In,Encode_Sp,System_Order);
              during:
              chu_jd=chu_jd-0.01;
              [PWMOUT,JD_Out,JD_Error,SGWY_Out] = Motor_XHZY(JD_In,Encode_Pos,YJ_In,Encode_Sp,System_Order);
            state Int4
              entry:
              chu_jd=0;
              [PWMOUT,JD_Out,JD_Error,SGWY_Out] = Motor_XHZY(JD_In,Encode_Pos,YJ_In,Encode_Sp,System_Order);
              during:
              [PWMOUT,JD_Out,JD_Error,SGWY_Out] = Motor_XHZY(JD_In,Encode_Pos,YJ_In,Encode_Sp,System_Order);
            state Int5
              entry:
              Motor_En=1;%电机失能
              PWMOUT=PWM_Value_Mid;
            state Int6
              entry:
              DCZD=1;%开启制动
            (default) -> Ready_Run.M_Run.Test_Mode.Limit_Up_Test.XHZY.Int
            Ready_Run.M_Run.Test_Mode.Limit_Up_Test.XHZY.Int -> Ready_Run.M_Run.Test_Mode.Limit_Up_Test.XHZY.Int1 : [after(0.5/Ts,tick)]
            Ready_Run.M_Run.Test_Mode.Limit_Up_Test.XHZY.Int1 -> Ready_Run.M_Run.Test_Mode.Limit_Up_Test.XHZY.Int2 : [Up_Limit==0]
                | %上限位开关低电平有效
            Ready_Run.M_Run.Test_Mode.Limit_Up_Test.XHZY.Int2 -> Ready_Run.M_Run.Test_Mode.Limit_Up_Test.XHZY.Int3 : [after(50,tick)]
            Ready_Run.M_Run.Test_Mode.Limit_Up_Test.XHZY.Int3 -> Ready_Run.M_Run.Test_Mode.Limit_Up_Test.XHZY.Int4 : [abs(chu_jd)<0.1]
            Ready_Run.M_Run.Test_Mode.Limit_Up_Test.XHZY.Int5 -> Ready_Run.M_Run.Test_Mode.Limit_Up_Test.XHZY.Int6 : [after(0.5/Ts,tick)]
            Ready_Run.M_Run.Test_Mode.Limit_Up_Test.XHZY.Int4 -> Ready_Run.M_Run.Test_Mode.Limit_Up_Test.XHZY.Int5 : [after(2/Ts,tick)]
          state HY
            %调试模式
            state Int6
              entry:
              DCZD=1;%开启制动
            state Int3
              entry:
              chu_jd=chu_jd-0.01;
              [PWMOUT,JD_Error,JD_Out] = Motor_HYDG(JD_In,Encode_Pos,System_Order,Encode_Sp);
              during:
              chu_jd=chu_jd-0.01;
              [PWMOUT,JD_Error,JD_Out] = Motor_HYDG(JD_In,Encode_Pos,System_Order,Encode_Sp);
            state Int
              en:
              Angle_Calculation=Angle_Calculation_HY(Encode_Pos);
              chu_jd=Angle_Calculation;
              DCZD=0;%解除制动
              Motor_En=0;%电机使能
              PWMOUT=PWM_Value_Mid;
              KG=1;
              KG_JD=uint8(0);
              KG_clc=~KG_clc;
            state Int5
              entry:
              Motor_En=1;%电机失能
              PWMOUT=PWM_Value_Mid;
            state Int4
              entry:
              chu_jd=0;
              [PWMOUT,JD_Error,JD_Out] = Motor_HYDG(JD_In,Encode_Pos,System_Order,Encode_Sp);
              during:
              [PWMOUT,JD_Error,JD_Out] = Motor_HYDG(JD_In,Encode_Pos,System_Order,Encode_Sp);
            state Int1
              entry:
              chu_jd=chu_jd+0.002;
              [PWMOUT,JD_Error,JD_Out] = Motor_HYDG(JD_In,Encode_Pos,System_Order,Encode_Sp);
              during:
              chu_jd=chu_jd+0.002;
              [PWMOUT,JD_Error,JD_Out] = Motor_HYDG(JD_In,Encode_Pos,System_Order,Encode_Sp);
            state Int2
              entry:
              chu_jd=chu_jd+0.002;
              [PWMOUT,JD_Error,JD_Out] = Motor_HYDG(JD_In,Encode_Pos,System_Order,Encode_Sp);
              during:
              chu_jd=chu_jd+0.002;
              [PWMOUT,JD_Error,JD_Out] = Motor_HYDG(JD_In,Encode_Pos,System_Order,Encode_Sp);
            (default) -> Ready_Run.M_Run.Test_Mode.Limit_Up_Test.HY.Int
            Ready_Run.M_Run.Test_Mode.Limit_Up_Test.HY.Int -> Ready_Run.M_Run.Test_Mode.Limit_Up_Test.HY.Int1 : [after(0.5/Ts,tick)]
            Ready_Run.M_Run.Test_Mode.Limit_Up_Test.HY.Int1 -> Ready_Run.M_Run.Test_Mode.Limit_Up_Test.HY.Int2 : [Up_Limit==0]
                | %上限位开关低电平有效
            Ready_Run.M_Run.Test_Mode.Limit_Up_Test.HY.Int2 -> Ready_Run.M_Run.Test_Mode.Limit_Up_Test.HY.Int3 : [after(50,tick)]
            Ready_Run.M_Run.Test_Mode.Limit_Up_Test.HY.Int3 -> Ready_Run.M_Run.Test_Mode.Limit_Up_Test.HY.Int4 : [abs(chu_jd)<0.1]
            Ready_Run.M_Run.Test_Mode.Limit_Up_Test.HY.Int5 -> Ready_Run.M_Run.Test_Mode.Limit_Up_Test.HY.Int6 : [after(0.5/Ts,tick)]
            Ready_Run.M_Run.Test_Mode.Limit_Up_Test.HY.Int4 -> Ready_Run.M_Run.Test_Mode.Limit_Up_Test.HY.Int5 : [after(2/Ts,tick)]
          (default) -> (junction 626)
          (junction 626) -> Ready_Run.M_Run.Test_Mode.Limit_Up_Test.XHHY [order 2] : [Motor_Num==3]
          (junction 626) -> Ready_Run.M_Run.Test_Mode.Limit_Up_Test.XHZY [order 1] : [Motor_Num==1]
          (junction 626) -> Ready_Run.M_Run.Test_Mode.Limit_Up_Test.HY [order 3] : [Motor_Num==2]
          Ready_Run.M_Run.Test_Mode.Limit_Up_Test.XHHY.Int6 -> (junction 627)
          Ready_Run.M_Run.Test_Mode.Limit_Up_Test.HY.Int6 -> (junction 627)
          Ready_Run.M_Run.Test_Mode.Limit_Up_Test.XHZY.Int6 -> (junction 627)
        state defult
          en:Open_Result=uint8(1);
          %开机状态位成功
          In_State=2;
        state Limit_Down_Test
          %电子下限位检测
          state HY
            %横摇灯杆电子下限位测试
            state Int
              en:
              Angle_Calculation=Angle_Calculation_HY(Encode_Pos);
              chu_jd=Angle_Calculation;
              DCZD=0;%解除制动
              Motor_En=0;%电机使能
              PWMOUT=PWM_Value_Mid;
              KG=1;
              KG_JD=uint8(0);
              KG_clc=~KG_clc;
            state Int1
              entry:
              chu_jd=chu_jd-0.002;
              [PWMOUT,JD_Error,JD_Out] = Motor_HYDG(JD_In,Encode_Pos,System_Order,Encode_Sp);
              during:
              chu_jd=chu_jd-0.002;
              [PWMOUT,JD_Error,JD_Out] = Motor_HYDG(JD_In,Encode_Pos,System_Order,Encode_Sp);
            state Int2
              entry:
              chu_jd=chu_jd-0.002;
              [PWMOUT,JD_Error,JD_Out] = Motor_HYDG(JD_In,Encode_Pos,System_Order,Encode_Sp);
              during:
              chu_jd=chu_jd-0.002;
              [PWMOUT,JD_Error,JD_Out] = Motor_HYDG(JD_In,Encode_Pos,System_Order,Encode_Sp);
            state Int3
              entry:
              chu_jd=chu_jd+0.01;
              [PWMOUT,JD_Error,JD_Out] = Motor_HYDG(JD_In,Encode_Pos,System_Order,Encode_Sp);
              during:
              chu_jd=chu_jd+0.01;
              [PWMOUT,JD_Error,JD_Out] = Motor_HYDG(JD_In,Encode_Pos,System_Order,Encode_Sp);
            state Int6
              entry:
              DCZD=1;%开启制动
            state Int4
              entry:
              chu_jd=0;
              [PWMOUT,JD_Error,JD_Out] = Motor_HYDG(JD_In,Encode_Pos,System_Order,Encode_Sp);
              during:
              [PWMOUT,JD_Error,JD_Out] = Motor_HYDG(JD_In,Encode_Pos,System_Order,Encode_Sp);
            state Int5
              entry:
              Motor_En=1;%电机失能
              PWMOUT=PWM_Value_Mid;
            (default) -> Ready_Run.M_Run.Test_Mode.Limit_Down_Test.HY.Int
            Ready_Run.M_Run.Test_Mode.Limit_Down_Test.HY.Int -> Ready_Run.M_Run.Test_Mode.Limit_Down_Test.HY.Int1 : [after(0.5/Ts,tick)]
            Ready_Run.M_Run.Test_Mode.Limit_Down_Test.HY.Int1 -> Ready_Run.M_Run.Test_Mode.Limit_Down_Test.HY.Int2 : [Down_Limit==0]
                | %上限位开关低电平有效
            Ready_Run.M_Run.Test_Mode.Limit_Down_Test.HY.Int2 -> Ready_Run.M_Run.Test_Mode.Limit_Down_Test.HY.Int3 : [after(50,tick)]
            Ready_Run.M_Run.Test_Mode.Limit_Down_Test.HY.Int3 -> Ready_Run.M_Run.Test_Mode.Limit_Down_Test.HY.Int4 : [abs(chu_jd)<0.1]
            Ready_Run.M_Run.Test_Mode.Limit_Down_Test.HY.Int5 -> Ready_Run.M_Run.Test_Mode.Limit_Down_Test.HY.Int6 : [after(0.5/Ts,tick)]
            Ready_Run.M_Run.Test_Mode.Limit_Down_Test.HY.Int4 -> Ready_Run.M_Run.Test_Mode.Limit_Down_Test.HY.Int5 : [after(2/Ts,tick)]
          state XHZY
            %下滑纵摇电子下限位测试
            state Int
              en:
              Angle_Calculation=Angle_Calculation_XH(Encode_Pos);
              chu_jd=Angle_Calculation;
              DCZD=0;%解除制动
              Motor_En=0;%电机使能
              PWMOUT=PWM_Value_Mid;
              KG=1;
              KG_JD=uint8(0);
              KG_YJ=uint8(0);
              KG_En=uint8(1);
              KG_clc=~KG_clc;
            state Int1
              entry:
              chu_jd=chu_jd-0.002;
              [PWMOUT,JD_Out,JD_Error,SGWY_Out] = Motor_XHZY(JD_In,Encode_Pos,YJ_In,Encode_Sp,System_Order);
              during:
              chu_jd=chu_jd-0.002;
              [PWMOUT,JD_Out,JD_Error,SGWY_Out] = Motor_XHZY(JD_In,Encode_Pos,YJ_In,Encode_Sp,System_Order);
            state Int2
              entry:
              chu_jd=chu_jd-0.002;
              [PWMOUT,JD_Out,JD_Error,SGWY_Out] = Motor_XHZY(JD_In,Encode_Pos,YJ_In,Encode_Sp,System_Order);
              during:
              chu_jd=chu_jd-0.002;
              [PWMOUT,JD_Out,JD_Error,SGWY_Out] = Motor_XHZY(JD_In,Encode_Pos,YJ_In,Encode_Sp,System_Order);
            state Int3
              entry:
              chu_jd=chu_jd+0.01;
              [PWMOUT,JD_Out,JD_Error,SGWY_Out] = Motor_XHZY(JD_In,Encode_Pos,YJ_In,Encode_Sp,System_Order);
              during:
              chu_jd=chu_jd+0.01;
              [PWMOUT,JD_Out,JD_Error,SGWY_Out] = Motor_XHZY(JD_In,Encode_Pos,YJ_In,Encode_Sp,System_Order);
            state Int6
              entry:
              DCZD=1;%开启制动
            state Int4
              entry:
              chu_jd=0;
              [PWMOUT,JD_Out,JD_Error,SGWY_Out] = Motor_XHZY(JD_In,Encode_Pos,YJ_In,Encode_Sp,System_Order);
              during:
              [PWMOUT,JD_Out,JD_Error,SGWY_Out] = Motor_XHZY(JD_In,Encode_Pos,YJ_In,Encode_Sp,System_Order);
            state Int5
              entry:
              Motor_En=1;%电机失能
              PWMOUT=PWM_Value_Mid;
            (default) -> Ready_Run.M_Run.Test_Mode.Limit_Down_Test.XHZY.Int
            Ready_Run.M_Run.Test_Mode.Limit_Down_Test.XHZY.Int -> Ready_Run.M_Run.Test_Mode.Limit_Down_Test.XHZY.Int1 : [after(0.5/Ts,tick)]
            Ready_Run.M_Run.Test_Mode.Limit_Down_Test.XHZY.Int1 -> Ready_Run.M_Run.Test_Mode.Limit_Down_Test.XHZY.Int2 : [Down_Limit==0]
                | %上限位开关低电平有效
            Ready_Run.M_Run.Test_Mode.Limit_Down_Test.XHZY.Int2 -> Ready_Run.M_Run.Test_Mode.Limit_Down_Test.XHZY.Int3 : [after(50,tick)]
            Ready_Run.M_Run.Test_Mode.Limit_Down_Test.XHZY.Int5 -> Ready_Run.M_Run.Test_Mode.Limit_Down_Test.XHZY.Int6 : [after(0.5/Ts,tick)]
            Ready_Run.M_Run.Test_Mode.Limit_Down_Test.XHZY.Int3 -> Ready_Run.M_Run.Test_Mode.Limit_Down_Test.XHZY.Int4 : [abs(chu_jd)<0.1]
            Ready_Run.M_Run.Test_Mode.Limit_Down_Test.XHZY.Int4 -> Ready_Run.M_Run.Test_Mode.Limit_Down_Test.XHZY.Int5 : [after(2/Ts,tick)]
          state XHHY
            %下滑横摇电子下限位测试
            state Int
              en:
              Angle_Calculation=Angle_Calculation_XH(Encode_Pos);
              chu_jd=Angle_Calculation;
              DCZD=0;%解除制动
              Motor_En=0;%电机使能
              PWMOUT=PWM_Value_Mid;
              KG=1;
              KG_JD=uint8(0);
              KG_En=uint8(1);
              KG_clc=~KG_clc;
            state Int1
              entry:
              chu_jd=chu_jd-0.002;
              [PWMOUT,JD_Out,JD_Error] = Motor_XHHY(JD_In,Encode_Pos,Encode_Sp,System_Order,SGWY_In);
              during:
              chu_jd=chu_jd-0.002;
              [PWMOUT,JD_Out,JD_Error] = Motor_XHHY(JD_In,Encode_Pos,Encode_Sp,System_Order,SGWY_In);
            state Int2
              entry:
              chu_jd=chu_jd-0.002;
              [PWMOUT,JD_Out,JD_Error] = Motor_XHHY(JD_In,Encode_Pos,Encode_Sp,System_Order,SGWY_In);
              during:
              chu_jd=chu_jd-0.002;
              [PWMOUT,JD_Out,JD_Error] = Motor_XHHY(JD_In,Encode_Pos,Encode_Sp,System_Order,SGWY_In);
            state Int3
              entry:
              chu_jd=chu_jd+0.01;
              [PWMOUT,JD_Out,JD_Error] = Motor_XHHY(JD_In,Encode_Pos,Encode_Sp,System_Order,SGWY_In);
              during:
              chu_jd=chu_jd+0.01;
              [PWMOUT,JD_Out,JD_Error] = Motor_XHHY(JD_In,Encode_Pos,Encode_Sp,System_Order,SGWY_In);
            state Int6
              entry:
              DCZD=1;%开启制动
            state Int4
              entry:
              chu_jd=0;
              [PWMOUT,JD_Out,JD_Error] = Motor_XHHY(JD_In,Encode_Pos,Encode_Sp,System_Order,SGWY_In);
              during:
              [PWMOUT,JD_Out,JD_Error] = Motor_XHHY(JD_In,Encode_Pos,Encode_Sp,System_Order,SGWY_In);
            state Int5
              entry:
              Motor_En=1;%电机失能
              PWMOUT=PWM_Value_Mid;
            (default) -> Ready_Run.M_Run.Test_Mode.Limit_Down_Test.XHHY.Int
            Ready_Run.M_Run.Test_Mode.Limit_Down_Test.XHHY.Int -> Ready_Run.M_Run.Test_Mode.Limit_Down_Test.XHHY.Int1 : [after(0.5/Ts,tick)]
            Ready_Run.M_Run.Test_Mode.Limit_Down_Test.XHHY.Int1 -> Ready_Run.M_Run.Test_Mode.Limit_Down_Test.XHHY.Int2 : [Down_Limit==0]
                | %上限位开关低电平有效
            Ready_Run.M_Run.Test_Mode.Limit_Down_Test.XHHY.Int2 -> Ready_Run.M_Run.Test_Mode.Limit_Down_Test.XHHY.Int3 : [after(50,tick)]
            Ready_Run.M_Run.Test_Mode.Limit_Down_Test.XHHY.Int3 -> Ready_Run.M_Run.Test_Mode.Limit_Down_Test.XHHY.Int4 : [abs(chu_jd)<0.1]
            Ready_Run.M_Run.Test_Mode.Limit_Down_Test.XHHY.Int5 -> Ready_Run.M_Run.Test_Mode.Limit_Down_Test.XHHY.Int6 : [after(0.5/Ts,tick)]
            Ready_Run.M_Run.Test_Mode.Limit_Down_Test.XHHY.Int4 -> Ready_Run.M_Run.Test_Mode.Limit_Down_Test.XHHY.Int5 : [after(2/Ts,tick)]
          (default) -> (junction 639)
          (junction 639) -> Ready_Run.M_Run.Test_Mode.Limit_Down_Test.XHHY [order 2] : [Motor_Num==3]
          (junction 639) -> Ready_Run.M_Run.Test_Mode.Limit_Down_Test.XHZY [order 1] : [Motor_Num==1]
          (junction 639) -> Ready_Run.M_Run.Test_Mode.Limit_Down_Test.HY [order 3] : [Motor_Num==2]
          Ready_Run.M_Run.Test_Mode.Limit_Down_Test.XHHY.Int6 -> (junction 640)
          Ready_Run.M_Run.Test_Mode.Limit_Down_Test.HY.Int6 -> (junction 640)
          Ready_Run.M_Run.Test_Mode.Limit_Down_Test.XHZY.Int6 -> (junction 640)
        state Elevation_Test
          %标定模式
          entry:
          DCZD=0;%解除制动
          Motor_En=0;%电机使能
          PWMOUT=PWM_Value_Mid;
          chu_jd=0;
          KG=1;
          state Int
            en:
            KG=1;
            KG_JD=uint8(0);
            KG_YJ=uint8(1);
            KG_En=uint8(1);
            KG_clc=~KG_clc;
          state Int1
            entry:
            [PWMOUT,JD_Out,JD_Error,SGWY_Out] = Motor_XHZY(JD_In,Encode_Pos,YJ_In,Encode_Sp,System_Order);
            during:
            [PWMOUT,JD_Out,JD_Error,SGWY_Out] = Motor_XHZY(JD_In,Encode_Pos,YJ_In,Encode_Sp,System_Order);
          state Int3
            entry:
            Motor_En=1;%电机失能
            PWMOUT=PWM_Value_Mid;
          state Int4
            entry:
            KG_YJ=uint8(0);
            [PWMOUT,JD_Out,JD_Error,SGWY_Out] = Motor_XHZY(JD_In,Encode_Pos,YJ_In,Encode_Sp,System_Order);
            during:
            [PWMOUT,JD_Out,JD_Error,SGWY_Out] = Motor_XHZY(JD_In,Encode_Pos,YJ_In,Encode_Sp,System_Order);
          (default) -> Ready_Run.M_Run.Test_Mode.Elevation_Test.Int
          Ready_Run.M_Run.Test_Mode.Elevation_Test.Int4 -> Ready_Run.M_Run.Test_Mode.Elevation_Test.Int3 : [JD_Error<0.1]
          Ready_Run.M_Run.Test_Mode.Elevation_Test.Int -> Ready_Run.M_Run.Test_Mode.Elevation_Test.Int1 : [after(0.5/Ts,tick)]
          Ready_Run.M_Run.Test_Mode.Elevation_Test.Int1 -> Ready_Run.M_Run.Test_Mode.Elevation_Test.Int4 : [Test_Mode ~= 4]
        (junction 640) -> Ready_Run.M_Run.Test_Mode.defult
        (junction 627) -> Ready_Run.M_Run.Test_Mode.defult
        Ready_Run.M_Run.Test_Mode.Elevation_Test.Int3 -> Ready_Run.M_Run.Test_Mode.defult
        (default) -> Ready_Run.M_Run.Test_Mode.defult
        Calibration -> Ready_Run.M_Run.Test_Mode.defult : [Test_Mode ~= 1]{DCZD=1;}
        Ready_Run.M_Run.Test_Mode.defult -> Elevation_Test [order 4] : [(Test_Mode == 4)&&(Motor_Num==1)]
        Ready_Run.M_Run.Test_Mode.defult -> Calibration [order 1] : [Test_Mode == 1]
        Ready_Run.M_Run.Test_Mode.defult -> Limit_Down_Test [order 3] : [Test_Mode == 3]
        Ready_Run.M_Run.Test_Mode.defult -> Limit_Up_Test [order 2] : [Test_Mode == 2]
        0 -> Close_Wait
      state Showing_Mode
        %检视模式
        entry:
        DCZD=0;%开电磁制动，低有效
        Open_Result=2;%开机状态位失败
        PWMOUT=PWM_Value_Mid;
        KG=0;
        state P4 [commented out]
          KG_clc=0;
        state P3 [commented out]
          KG_clc=1;
        state RUN
          state GXDY_SJ_BJ [parallel]
            during:JD_Vary = COM_Error(JD_In);
            settings: executionOrder=3
            state Defult
            state p1
              entry: can1_i=uint16(0);%计数器置零
              du:Flag_GXDY_Error=uint8(1);
              %惯性单元正常
            state p4
              en:can1_i= uint16(1);
              du:can1_i = can1_i + 1;
            note: CAN收到数据，但是数据不对,
                | 大于速度最大值
            state p3
              %0代表正常，1代表错误
              entry: can1_i= uint16(0);
              %Motor_En=uint8(1);%电机失能
              Flag_GXDY_Error=uint8(0);
              %惯性单元通讯故障
            state p2
              en:can1_i=uint16(1);
              du:can1_i = can1_i + 1;
            (default) -> Ready_Run.M_Run.Showing_Mode.RUN.GXDY_SJ_BJ.Defult
            Ready_Run.M_Run.Showing_Mode.RUN.GXDY_SJ_BJ.Defult -> Ready_Run.M_Run.Showing_Mode.RUN.GXDY_SJ_BJ.p1 : [Open_Result==1&&GXDY_State==0]
                | %开机成功且惯性单元打开
            Ready_Run.M_Run.Showing_Mode.RUN.GXDY_SJ_BJ.p4 -> Ready_Run.M_Run.Showing_Mode.RUN.GXDY_SJ_BJ.p1 [order 2] : [can1_i>=2/Ts]
            Ready_Run.M_Run.Showing_Mode.RUN.GXDY_SJ_BJ.p4 -> Ready_Run.M_Run.Showing_Mode.RUN.GXDY_SJ_BJ.p3 [order 1] : [JD_Vary>JD_Max]
            Ready_Run.M_Run.Showing_Mode.RUN.GXDY_SJ_BJ.p3 -> Ready_Run.M_Run.Showing_Mode.RUN.GXDY_SJ_BJ.p4 : [JD_Vary<=JD_Max]
            Ready_Run.M_Run.Showing_Mode.RUN.GXDY_SJ_BJ.p1 -> Ready_Run.M_Run.Showing_Mode.RUN.GXDY_SJ_BJ.p2 : [JD_Vary>JD_Max]
                | %速度大于最大值
            Ready_Run.M_Run.Showing_Mode.RUN.GXDY_SJ_BJ.p2 -> Ready_Run.M_Run.Showing_Mode.RUN.GXDY_SJ_BJ.p1 [order 1] : [JD_Vary<=JD_Max]
            Ready_Run.M_Run.Showing_Mode.RUN.GXDY_SJ_BJ.p2 -> Ready_Run.M_Run.Showing_Mode.RUN.GXDY_SJ_BJ.p3 [order 2] : [can1_i>=2/Ts]%2S
          state GXDY_COM_GZ [parallel]
            settings: executionOrder=1
            state Defult
            state r2
              entry:
              Flag_GXDY_IT=0;%故障
            state p7
              entry:
              GXDY_i=0;%计数器置零
              Flag_GXDY_IT=1;%正常
            state p6
              %1代表正常，0代表错误
              entry:
              Flag_GXDY_IT=0;%故障
              %Motor_En=1;%电机失能
            state p5
              en:GXDY_i=1;
              du:GXDY_i = GXDY_i + 1;
            Ready_Run.M_Run.Showing_Mode.RUN.GXDY_COM_GZ.Defult -> (junction 564) [order 2] : [Open_Result==1]
                | %开机成功
            (junction 564) -> (junction 565) : after(10/Ts,tick)
            (default) -> Ready_Run.M_Run.Showing_Mode.RUN.GXDY_COM_GZ.Defult
            Ready_Run.M_Run.Showing_Mode.RUN.GXDY_COM_GZ.Defult -> Ready_Run.M_Run.Showing_Mode.RUN.GXDY_COM_GZ.p7 [order 1] : [Open_Result==1&&GXDY_State==0]
                | %开机成功且惯性单元打开
            (junction 565) -> Ready_Run.M_Run.Showing_Mode.RUN.GXDY_COM_GZ.r2 : [GXDY_State==1]
            Ready_Run.M_Run.Showing_Mode.RUN.GXDY_COM_GZ.p7 -> Ready_Run.M_Run.Showing_Mode.RUN.GXDY_COM_GZ.p5 : [GXDY_IT_In==0]
            Ready_Run.M_Run.Showing_Mode.RUN.GXDY_COM_GZ.p5 -> Ready_Run.M_Run.Showing_Mode.RUN.GXDY_COM_GZ.p7 [order 1] : [GXDY_IT_In==1]
            Ready_Run.M_Run.Showing_Mode.RUN.GXDY_COM_GZ.p5 -> Ready_Run.M_Run.Showing_Mode.RUN.GXDY_COM_GZ.p6 [order 2] : [GXDY_i>=uint16(3/Ts)]%3S
          state Limit_Check [parallel]
            settings: executionOrder=4
            state p1
              entry:
              Flag_Down_limit=1;
              Flag_Up_limit=1;
              Flag_Up_GZ_limit=1;
              Flag_Down_GZ_limit=1;
            state defult
            state p2
              entry:Flag_Up_limit=0;
            state p3
              entry: Flag_Down_limit=0;
            (default) -> Ready_Run.M_Run.Showing_Mode.RUN.Limit_Check.defult
            Ready_Run.M_Run.Showing_Mode.RUN.Limit_Check.defult -> Ready_Run.M_Run.Showing_Mode.RUN.Limit_Check.p1 : [after(1/Ts,tick)]
            Ready_Run.M_Run.Showing_Mode.RUN.Limit_Check.p1 -> Ready_Run.M_Run.Showing_Mode.RUN.Limit_Check.p2 [order 1] : [Up_Limit==0]
            Ready_Run.M_Run.Showing_Mode.RUN.Limit_Check.p2 -> Ready_Run.M_Run.Showing_Mode.RUN.Limit_Check.p1 : [Up_Limit==1]
            Ready_Run.M_Run.Showing_Mode.RUN.Limit_Check.p1 -> Ready_Run.M_Run.Showing_Mode.RUN.Limit_Check.p3 [order 2] : [Down_Limit==0]
            Ready_Run.M_Run.Showing_Mode.RUN.Limit_Check.p3 -> Ready_Run.M_Run.Showing_Mode.RUN.Limit_Check.p1 : [Down_Limit==1]
          state Algorithm [parallel]
            settings: executionOrder=2
            state Defualt
              en:chu_jd=0;
              KG=0;
              Motor_En=0;
            state XHHY
              state Defualt
                entry:
                %en:KG_En=uint8(0);KG_JD=uint8(1);KG_YJ=uint8(1);
                KG_En=uint8(1);KG_JD=uint8(0);KG_clc=~KG_clc;
                during:[PWMOUT,JD_Out,JD_Error] = Motor_XHHY(JD_In,Encode_Pos,Encode_Sp,System_Order,SGWY_In);
              state Sleeping_protect_2
                entry:
                DCZD=1;%关电磁制动
                exit:
                DCZD=0;%开电磁制动
              state XHHY_Error
                en:Motor_En=uint8(1);%关电机
              state Sleeping_protect_1
                entry:
                Motor_En=1;%关电机
                PWMOUT=PWM_Value_Mid;
              state XHHY_Wait
                en:Open_Result=uint8(1);
                %开机状态位成功
                In_State=2;
                KG_En=uint8(1);KG_clc=~KG_clc;
                during:[PWMOUT,JD_Out,JD_Error] = Motor_XHHY(JD_In,Encode_Pos,Encode_Sp,System_Order,SGWY_In);
                %PWMOUT=2500;
              state XHHY_Run
                en:KG_En=uint8(0);KG_JD=uint8(1);KG_clc=~KG_clc;
                %外部接口
                during:KG_JD=uint8(1);
                Angle=Showing(Showing_Angle,Showing_T);
                chu_jd=Angle;
                [PWMOUT,JD_Out,JD_Error] = Motor_XHHY(JD_In,Encode_Pos,Encode_Sp,System_Order,SGWY_In);
              state Sleeping_protect_3
                entry:
                Motor_En=0;%开电机
              (default) -> Ready_Run.M_Run.Showing_Mode.RUN.Algorithm.XHHY.Defualt
              Ready_Run.M_Run.Showing_Mode.RUN.Algorithm.XHHY.Defualt -> Ready_Run.M_Run.Showing_Mode.RUN.Algorithm.XHHY.XHHY_Wait [order 1] : [abs(Encode_Pos)<=Encode_Pos_Zero]
              Ready_Run.M_Run.Showing_Mode.RUN.Algorithm.XHHY.Defualt -> Ready_Run.M_Run.Showing_Mode.RUN.Algorithm.XHHY.XHHY_Error [order 2] : [after(10/Ts,tick)]
              Ready_Run.M_Run.Showing_Mode.RUN.Algorithm.XHHY.Sleeping_protect_1 -> Ready_Run.M_Run.Showing_Mode.RUN.Algorithm.XHHY.Sleeping_protect_2 : [after(0.5/Ts,tick)]
              Ready_Run.M_Run.Showing_Mode.RUN.Algorithm.XHHY.Sleeping_protect_2 -> Ready_Run.M_Run.Showing_Mode.RUN.Algorithm.XHHY.Sleeping_protect_3 : [System_Order==5]
              Ready_Run.M_Run.Showing_Mode.RUN.Algorithm.XHHY.XHHY_Run -> Ready_Run.M_Run.Showing_Mode.RUN.Algorithm.XHHY.Sleeping_protect_1 [order 2] : [System_Order==4]
              Ready_Run.M_Run.Showing_Mode.RUN.Algorithm.XHHY.Sleeping_protect_3 -> Ready_Run.M_Run.Showing_Mode.RUN.Algorithm.XHHY.XHHY_Run : [after(0.5/Ts,tick)]
              Ready_Run.M_Run.Showing_Mode.RUN.Algorithm.XHHY.XHHY_Wait -> Ready_Run.M_Run.Showing_Mode.RUN.Algorithm.XHHY.XHHY_Run : [GXDY_State==0]
                  | %惯性单元拉低
            state HY
              state Sleeping_protect_3
                entry:
                Motor_En=0;%开电机
              state Sleeping_protect_2
                entry:
                DCZD=1;%关电磁制动
                exit:
                DCZD=0;%开电磁制动
              state Defualt1
                entry:
                KG_JD=uint8(0);
                during:[PWMOUT,JD_Error,JD_Out] = Motor_HYDG(JD_In,Encode_Pos,System_Order,Encode_Sp);
              state XHHY_Error
                en:Motor_En=uint8(1);%关电机
              state XHHY_Wait
                en:Open_Result=uint8(1);
                %开机状态位成功
                In_State=2;
                during:[PWMOUT,JD_Error,JD_Out] = Motor_HYDG(JD_In,Encode_Pos,System_Order,Encode_Sp);
                %PWMOUT=2500;
              state XHHY_Run
                en:KG_JD=uint8(1);
                %外部接口
                during:%[PWMOUT,JD_Error,JD_Out] = Motor_HYDG1(JD_In,Encode_Pos,System_Order):
                Angle=Showing(Showing_Angle,Showing_T);
                chu_jd=Angle;
                [PWMOUT,JD_Error,JD_Out] = Motor_HYDG1(JD_In,Encode_Pos,System_Order);
              state Sleeping_protect_1
                entry:
                Motor_En=1;%关电机
                PWMOUT=PWM_Value_Mid;
              (default) -> Ready_Run.M_Run.Showing_Mode.RUN.Algorithm.HY.Defualt1
              Ready_Run.M_Run.Showing_Mode.RUN.Algorithm.HY.Sleeping_protect_1 -> Ready_Run.M_Run.Showing_Mode.RUN.Algorithm.HY.Sleeping_protect_2 : [after(0.5/Ts,tick)]
              Ready_Run.M_Run.Showing_Mode.RUN.Algorithm.HY.Defualt1 -> Ready_Run.M_Run.Showing_Mode.RUN.Algorithm.HY.XHHY_Wait [order 1] : [abs(Encode_Pos)<=Encode_Pos_Zero]
              Ready_Run.M_Run.Showing_Mode.RUN.Algorithm.HY.Defualt1 -> Ready_Run.M_Run.Showing_Mode.RUN.Algorithm.HY.XHHY_Error [order 2] : [after(10/Ts,tick)]
              Ready_Run.M_Run.Showing_Mode.RUN.Algorithm.HY.Sleeping_protect_2 -> Ready_Run.M_Run.Showing_Mode.RUN.Algorithm.HY.Sleeping_protect_3 : [System_Order==5]
              Ready_Run.M_Run.Showing_Mode.RUN.Algorithm.HY.XHHY_Run -> Ready_Run.M_Run.Showing_Mode.RUN.Algorithm.HY.Sleeping_protect_1 [order 2] : [System_Order==4]
              Ready_Run.M_Run.Showing_Mode.RUN.Algorithm.HY.Sleeping_protect_3 -> Ready_Run.M_Run.Showing_Mode.RUN.Algorithm.HY.XHHY_Run : [after(0.5/Ts,tick)]
              Ready_Run.M_Run.Showing_Mode.RUN.Algorithm.HY.XHHY_Wait -> (junction 601) : after(5,tick)
              (junction 601) -> Ready_Run.M_Run.Showing_Mode.RUN.Algorithm.HY.XHHY_Run : [GXDY_State==0]
                  | %惯性单元拉低
            state XHZY
              state Sleeping_protect_3
                entry:
                Motor_En=0;%开电机
              state Defualt
                entry:
                %en:KG_En=uint8(0);KG_JD=uint8(1);KG_YJ=uint8(1);
                KG_En=uint8(1);KG_JD=uint8(0);KG_YJ=uint8(0);KG_clc=0;
                during:[PWMOUT,JD_Out,JD_Error,SGWY_Out] = Motor_XHZY(JD_In,Encode_Pos,YJ_In,Encode_Sp,System_Order);
              state XHZY_Error
                en:Motor_En=1;%电机失能
              state XHZY_Wait
                en:Open_Result=1;
                %开机状态位成功
                In_State=2;
                KG_En=uint8(1);KG_clc=1;
                during:[PWMOUT,JD_Out,JD_Error,SGWY_Out] = Motor_XHZY(JD_In,Encode_Pos,YJ_In,Encode_Sp,System_Order);
                %PWMOUT=2500;
              state XHZY_Run
                en:KG_En=uint8(0);KG_JD=uint8(1);KG_YJ=uint8(1);KG_clc=0;
                %KG_YJ=uint8(1);%接入外部接口
                during:
                Angle=Showing(Showing_Angle,Showing_T);
                chu_jd=Angle;
                [PWMOUT,JD_Out,JD_Error,SGWY_Out] = Motor_XHZY(JD_In,Encode_Pos,YJ_In,Encode_Sp,System_Order);
              state Sleeping_protect_1
                entry:
                Motor_En=1;%关电机
                PWMOUT=PWM_Value_Mid;
              state Sleeping_protect_2
                entry:
                DCZD=1;%关电磁制动
                exit:
                DCZD=0;%开电磁制动
              (default) -> Ready_Run.M_Run.Showing_Mode.RUN.Algorithm.XHZY.Defualt
              Ready_Run.M_Run.Showing_Mode.RUN.Algorithm.XHZY.Defualt -> Ready_Run.M_Run.Showing_Mode.RUN.Algorithm.XHZY.XHZY_Wait [order 2] : [abs(Encode_Pos)<=Encode_Pos_Zero]
              Ready_Run.M_Run.Showing_Mode.RUN.Algorithm.XHZY.Defualt -> Ready_Run.M_Run.Showing_Mode.RUN.Algorithm.XHZY.XHZY_Error [order 1] : [after(15/Ts,tick)]%等待15s
              Ready_Run.M_Run.Showing_Mode.RUN.Algorithm.XHZY.Sleeping_protect_1 -> Ready_Run.M_Run.Showing_Mode.RUN.Algorithm.XHZY.Sleeping_protect_2 : [after(0.5/Ts,tick)]
              Ready_Run.M_Run.Showing_Mode.RUN.Algorithm.XHZY.Sleeping_protect_2 -> Ready_Run.M_Run.Showing_Mode.RUN.Algorithm.XHZY.Sleeping_protect_3 : [System_Order==5]
              Ready_Run.M_Run.Showing_Mode.RUN.Algorithm.XHZY.XHZY_Run -> Ready_Run.M_Run.Showing_Mode.RUN.Algorithm.XHZY.Sleeping_protect_1 [order 1] : [System_Order==4]
              Ready_Run.M_Run.Showing_Mode.RUN.Algorithm.XHZY.XHZY_Wait -> (junction 612) : after(5,tick)
              Ready_Run.M_Run.Showing_Mode.RUN.Algorithm.XHZY.Sleeping_protect_3 -> Ready_Run.M_Run.Showing_Mode.RUN.Algorithm.XHZY.XHZY_Run : [after(0.5/Ts,tick)]
              (junction 612) -> (junction 613) [order 2] : [System_Order==3]
              (junction 612) -> Ready_Run.M_Run.Showing_Mode.RUN.Algorithm.XHZY.XHZY_Run [order 1] : [GXDY_State==0]
                  | %惯性单元拉低
              Ready_Run.M_Run.Showing_Mode.RUN.Algorithm.XHZY.XHZY_Run -> (junction 613) [order 2] : [System_Order==3]
            (default) -> Ready_Run.M_Run.Showing_Mode.RUN.Algorithm.Defualt
            Ready_Run.M_Run.Showing_Mode.RUN.Algorithm.Defualt -> Ready_Run.M_Run.Showing_Mode.RUN.Algorithm.XHHY [order 1] : [Motor_Num==3]
            Ready_Run.M_Run.Showing_Mode.RUN.Algorithm.Defualt -> Ready_Run.M_Run.Showing_Mode.RUN.Algorithm.XHZY [order 3] : [Motor_Num==1]
            Ready_Run.M_Run.Showing_Mode.RUN.Algorithm.Defualt -> Ready_Run.M_Run.Showing_Mode.RUN.Algorithm.HY [order 2] : [Motor_Num==2]
            Ready_Run.M_Run.Showing_Mode.RUN.Algorithm.HY.XHHY_Run -> (junction 580) [order 1] : [System_Order==3]
            (junction 613) -> (junction 580)
            Ready_Run.M_Run.Showing_Mode.RUN.Algorithm.XHHY.XHHY_Run -> (junction 580) [order 1] : [System_Order==3]
          (default) -> Ready_Run.M_Run.Showing_Mode.RUN.Algorithm
        state Start
        Ready_Run.M_Run.Showing_Mode.P3 -> ? [commented out] : [after(1/Ts,tick)]
        (default) -> Ready_Run.M_Run.Showing_Mode.P3 [commented out] : [KG_clc == 0]
        (default) -> Ready_Run.M_Run.Showing_Mode.P4 [commented out] : [KG_clc > 0]
        Ready_Run.M_Run.Showing_Mode.P4 -> ? [commented out] : [after(1/Ts,tick)]
        (default) -> Start
        Start -> Ready_Run.M_Run.Showing_Mode.RUN : [after(1/Ts,tick)]
      state Close
        state Algorithm
          state HYDG_Close
            en:KG_JD=uint8(0);KG_clc=~KG_clc;
            state XHZY_Error
              en:Motor_En=1;%电机失能
            state Defualt
              en:
              chu_jd=0;
              du:
              [PWMOUT,JD_Error,JD_Out] = Motor_HYDG(JD_In,Encode_Pos,System_Order,Encode_Sp);
            state XHZY_Close
              en:Open_Result=2;%关机成功
              In_State=3;
              DCZD=1;%电池只懂引脚拉高，关电磁制动，低有效
            state XHZY_Close1
              en:Motor_En=1;%电机失能
              PWMOUT=PWM_Value_Mid;
            state Int
              en:
              Angle_Calculation=Angle_Calculation_HY(Encode_Pos);
              chu_jd=Angle_Calculation;
              KG=1;
              KG_JD=uint8(0);
              KG_clc=~KG_clc;
            state Int1
              en:
              chu_jd=chu_jd+0.01;
              [PWMOUT,JD_Error,JD_Out] = Motor_HYDG(JD_In,Encode_Pos,System_Order,Encode_Sp);
              du:
              chu_jd=chu_jd+0.01;
              [PWMOUT,JD_Error,JD_Out] = Motor_HYDG(JD_In,Encode_Pos,System_Order,Encode_Sp);
            state Int2
              en:
              chu_jd=chu_jd-0.01;
              [PWMOUT,JD_Error,JD_Out] = Motor_HYDG(JD_In,Encode_Pos,System_Order,Encode_Sp);
              du:
              chu_jd=chu_jd-0.01;
              [PWMOUT,JD_Error,JD_Out] = Motor_HYDG(JD_In,Encode_Pos,System_Order,Encode_Sp);
            (default) -> Ready_Run.M_Run.Close.Algorithm.HYDG_Close.Int
            Ready_Run.M_Run.Close.Algorithm.HYDG_Close.Int -> Ready_Run.M_Run.Close.Algorithm.HYDG_Close.Int1 [order 1] : [chu_jd < 0]
            Ready_Run.M_Run.Close.Algorithm.HYDG_Close.Int -> Ready_Run.M_Run.Close.Algorithm.HYDG_Close.Int2 [order 2] : [chu_jd > 0]
            Ready_Run.M_Run.Close.Algorithm.HYDG_Close.Int -> Ready_Run.M_Run.Close.Algorithm.HYDG_Close.Defualt [order 3] : [chu_jd == 0]
            Ready_Run.M_Run.Close.Algorithm.HYDG_Close.Int1 -> Ready_Run.M_Run.Close.Algorithm.HYDG_Close.Defualt : [abs(chu_jd)<0.1]
            Ready_Run.M_Run.Close.Algorithm.HYDG_Close.Int2 -> Ready_Run.M_Run.Close.Algorithm.HYDG_Close.Defualt : [abs(chu_jd)<0.1]
            Ready_Run.M_Run.Close.Algorithm.HYDG_Close.Defualt -> Ready_Run.M_Run.Close.Algorithm.HYDG_Close.XHZY_Close1 [order 1] : [abs(Encode_Pos)<=Encode_Pos_Zero]
            Ready_Run.M_Run.Close.Algorithm.HYDG_Close.Defualt -> Ready_Run.M_Run.Close.Algorithm.HYDG_Close.XHZY_Error [order 2] : [after(2/Ts,tick)]%等待2s，查看关机是否成功
            Ready_Run.M_Run.Close.Algorithm.HYDG_Close.XHZY_Error -> Ready_Run.M_Run.Close.Algorithm.HYDG_Close.XHZY_Close1
            Ready_Run.M_Run.Close.Algorithm.HYDG_Close.XHZY_Close1 -> Ready_Run.M_Run.Close.Algorithm.HYDG_Close.XHZY_Close : [after(0.5/Ts,tick)]
          state XHHY_Close
            entry:KG_En=1;KG_JD=0;KG_clc=~KG_clc;
            during:[PWMOUT,JD_Out,JD_Error] = Motor_XHHY(JD_In,Encode_Pos,Encode_Sp,System_Order,SGWY_In);
            state XHZY_Error
              en:Motor_En=1;%电机失能
            state Defualt
            state XHZY_Close
              en:Open_Result=2;%关机成功
              In_State=3;
              DCZD=1;%电池只懂引脚拉高，关电磁制动，低有效
            state XHZY_Close1
              en:Motor_En=1;%电机失能
              PWMOUT=PWM_Value_Mid;
            (default) -> Ready_Run.M_Run.Close.Algorithm.XHHY_Close.Defualt
            Ready_Run.M_Run.Close.Algorithm.XHHY_Close.Defualt -> Ready_Run.M_Run.Close.Algorithm.XHHY_Close.XHZY_Error [order 1] : [after(10/Ts,tick)]%等待10s，查看关机是否成功
            Ready_Run.M_Run.Close.Algorithm.XHHY_Close.Defualt -> Ready_Run.M_Run.Close.Algorithm.XHHY_Close.XHZY_Close1 [order 2] : [abs(Encode_Pos)<=Encode_Pos_Zero]
            Ready_Run.M_Run.Close.Algorithm.XHHY_Close.XHZY_Error -> Ready_Run.M_Run.Close.Algorithm.XHHY_Close.XHZY_Close1
            Ready_Run.M_Run.Close.Algorithm.XHHY_Close.XHZY_Close1 -> Ready_Run.M_Run.Close.Algorithm.XHHY_Close.XHZY_Close : [after(0.5/Ts,tick)]
          state XHZY_Close
            entry:KG_En=1;KG_JD=0;KG_YJ=0;KG_clc=~KG_clc;chu_jd=0;
            during:[PWMOUT,JD_Out,JD_Error,SGWY_Out] = Motor_XHZY(JD_In,Encode_Pos,YJ_In,Encode_Sp,System_Order);
            state XHZY_Close
              en:Motor_En=1;%电机失能
              PWMOUT=PWM_Value_Mid;
            state XHZY_Error
              en:Motor_En=1;%电机失能
            state Defualt
            state XHZY_Close1
              en:Open_Result=2;%关机成功
              In_State=3;
              DCZD=1;%电池只懂引脚拉高，关电磁制动，低有效
            Ready_Run.M_Run.Close.Algorithm.XHZY_Close.Defualt -> Ready_Run.M_Run.Close.Algorithm.XHZY_Close.XHZY_Error [order 2] : [after(10/Ts,tick)]%等待10s，查看关机是否成功
            Ready_Run.M_Run.Close.Algorithm.XHZY_Close.XHZY_Error -> Ready_Run.M_Run.Close.Algorithm.XHZY_Close.XHZY_Close
            (default) -> Ready_Run.M_Run.Close.Algorithm.XHZY_Close.Defualt
            Ready_Run.M_Run.Close.Algorithm.XHZY_Close.Defualt -> Ready_Run.M_Run.Close.Algorithm.XHZY_Close.XHZY_Close [order 1] : [abs(Encode_Pos)<=Encode_Pos_Zero]
            Ready_Run.M_Run.Close.Algorithm.XHZY_Close.XHZY_Close -> Ready_Run.M_Run.Close.Algorithm.XHZY_Close.XHZY_Close1 : [after(0.5/Ts,tick)]
          (junction 459) -> Ready_Run.M_Run.Close.Algorithm.XHZY_Close [order 1] : [Motor_Num==1]
          (junction 459) -> HYDG_Close [order 2] : [Motor_Num==2]
          (junction 459) -> XHHY_Close [order 3] : [Motor_Num==3]
        state Close_Wait
          entry:
          DCZD=0;%解除制动
          Motor_En=0;%电机使能
          PWMOUT=PWM_Value_Mid;
        Close_Wait -> (junction 459) : [after(0.5/Ts,tick)]
      (junction 268) -> Test_Mode [order 3] : [Working_Mode == 1]
      (default) -> Initialize
      (junction 268) -> Showing_Mode [order 2] : [Working_Mode == 2]
      Close -> (junction 268) [order 1] : [System_Order==2]
      (junction 268) -> Normal_Mode [order 1] : [Working_Mode == 3]
      Close -> Initialize [order 2] : [System_Order==1]
      (junction 580) -> Close_Wait
      (junction 511) -> Close_Wait
      Test_Mode -> Close_Wait : [System_Order==3]
      Check_Reset -> (junction 268) : [(Ini_Result==1)&&(System_Order==2)]
          | %代表初始化成功，接收开机指令
    state Temp_check [parallel]
      du:Flag_Temp_Up=Temp_Up_Check(Temp_In,Temp_Up_Limit);
      Flag_Temp_Down=Temp_Down_Check(Temp_In,Temp_Down_Limit);
      settings: executionOrder=2
    state ZHI_S_D [parallel]
      %指示灯
      during:[QDQ_HY,QDQ_XH] = BJ(In_State,QDQ_BJ)
      settings: executionOrder=4
      state defult
        en:QDQ_BJ=1;
        Alarm_Cunt=1;
      state QDQ_GZ
        en:QDQ_BJ=3;
        Alarm_Cunt=3;
        Motor_En=1;
        du:Alarm_Cunt=1;
      state QDQ_BJ
        en:QDQ_BJ=2;
        Alarm_Cunt=2;
        du:Alarm_Cunt=1;
      (default) -> Ready_Run.ZHI_S_D.defult
      Ready_Run.ZHI_S_D.defult -> QDQ_BJ [order 1] : [Flag_Cur==0||Flag_Temp_Up==0||(Flag_Up_limit==0)||(Flag_Down_limit==0)||Flag_GXDY_Error==0]
      QDQ_BJ -> Ready_Run.ZHI_S_D.defult [order 2] : [Flag_Cur==1&&Flag_Temp_Up==1&&(Flag_Up_limit==1)&&(Flag_Down_limit==1)&&Flag_GXDY_Error==1]
      Ready_Run.ZHI_S_D.defult -> QDQ_GZ [order 2] : [(Flag_GZ_Cur==0)||(Flag_Motor_Error==0)||Flag_Temp_Down==0||Flag_Enc_Error==0||Flag_GXDY_IT==0]
      QDQ_BJ -> QDQ_GZ [order 1] : [(Flag_Up_GZ_limit==0)||(Flag_Down_GZ_limit==0)||(Flag_GZ_Cur==0)||(Flag_Motor_Error==0)||Flag_Temp_Down==0||Flag_Enc_Error==0||Flag_GXDY_IT==0]
  state [PWMOUT,JD_Out,JD_Error] = Motor_XHHY(JD_In,Encode_Pos,Encode_Sp,Slect_port,SGWY_In) [function]
  state y=Temp_Up_Check(In1,In2) [function]
    (default) -> (junction 344)
    (junction 344) -> (junction 345) [order 1] : [In1>=In2]
    (junction 344) -> (junction 346) [order 2] : {y=uint8(1);}
    (junction 345) -> (junction 347) : {y=uint8(0);}
    (junction 347) -> (junction 346)
    (junction 346) -> (junction 348)
  state PWMOUT = Open_Motor(Encode_Sp) [function]
  state [PWMOUT,JD_Error,JD_Out] = Motor_HYDG(JD_In,Encode_Pos,Slect_port,Encode_Sp) [function]
  state y=Temp_Down_Check(In1,In2) [function]
    (default) -> (junction 403)
    (junction 403) -> (junction 404) [order 1] : [In1<=In2]
    (junction 403) -> (junction 405) [order 2] : {y=uint8(1);}
    (junction 404) -> (junction 406) : {y=uint8(0);}
    (junction 406) -> (junction 405)
    (junction 405) -> (junction 407)
  state [PWMOUT,JD_Out,JD_Error,SGWY_Out] = Motor_XHZY(JD_In,Encode_Pos,YJ_In,Encode_Sp,Slect_port) [function]
  state [Out1,Out2] = BJ(x,y) [function]
  state Out = COM_Error(In) [function]
  state [PWMOUT,JD_Error,JD_Out] = Motor_HYDG1(JD_In,Encode_Pos,Slect_port) [function]
  state Angle=Showing(Showing_Angle,Showing_T) [function]
  state [JD_Error,JD_Out,SGWY_Out] = Angle_Calculation(JD_In,Motor_Num,Encode_Pos,SGWY_In) [function] [commented out]
  state Angle_Calculation = Angle_Calculation_XH(Encode_Pos) [function]
  state Angle_Calculation = Angle_Calculation_HY(Encode_Pos) [function]
  Ready -> Ready_Run : [System_Order==uint8(1)]
  (default) -> Ready
  data: JD_In function_input int32 size=1; Encode_Pos function_input int32 size=1; Encode_Sp function_input int32 size=1; PWMOUT function_output double; JD_Out function_output double; JD_Error function_output double; Slect_port function_input uint8 size=1; SGWY_In function_input int32 size=1; y function_output uint8 size=1; In1 function_input uint16 size=1; In2 function_input uint16 size=1; Encode_Sp function_input int32 size=1; PWMOUT function_output double; JD_In function_input int32 size=1; Encode_Pos function_input int32 size=1; PWMOUT function_output double; JD_Error function_output double; JD_Out function_output double; Slect_port function_input uint8 size=1; Encode_Sp function_input int32 size=1; y function_output uint8 size=1; In1 function_input uint16 size=1; In2 function_input uint16 size=1; JD_In function_input int32 size=1; Encode_Pos function_input int32 size=1; YJ_In function_input int32 size=1; Encode_Sp function_input int32 size=1; PWMOUT function_output double; JD_Out function_output double; JD_Error function_output double; Slect_port function_input uint8 size=1; SGWY_Out function_output int32; x function_input uint8; y function_input double; Out1 function_output boolean; Out2 function_output boolean; In1 function_input uint8 size=1; In2 function_input uint8 size=1; y function_output uint8 size=1; In3 function_input double; In function_input double; Out function_output double; JD_In function_input int32 size=1; Encode_Pos function_input int32 size=1; PWMOUT function_output double; JD_Error function_output double; JD_Out function_output double; Slect_port function_input uint8 size=1; Showing_Angle function_input double; Showing_T function_input double; Angle function_output double; JD_In function_input double size=1; JD_Error function_output double size=1; Motor_Num function_input double size=1; Encode_Pos function_input double size=1; SGWY_In function_input double size=1; JD_Out function_output double size=1; SGWY_Out function_output double size=1; Encode_Pos function_input int32 size=1; Angle_Calculation function_output double; Encode_Pos function_input int32 size=1; Angle_Calculation function_output double; System_Order input uint8 size=1; Cur_Limit local uint32 size=1; Temp_Up_Limit local uint32 size=1; Ini_Result output uint8 size=1; PWM_Value_Up local uint16 size=1; PWM_Value_Down local uint16 size=1; PWM_Value_Mid local uint16 size=1; Encode_Sp_Min local uint32 size=1; Encode_Pos1 local int32 size=1; Encode_Pos2 local int32 size=1; Encode_Pos3 local int32 size=1; Encode_Pos_Zero local uint32 size=1; Ts local double size=1; JD_Max local uint32 size=1; Encode_Pos_Min local uint32 size=1; Encode_Sp_Max local uint32 size=1; cur_i local uint16 size=1; Flag_Cur output uint8 size=1; Cur_In input uint32 size=1; Motor_En output boolean size=1; Temp_In input uint32 size=1; Flag_Temp_Up output uint8 size=1; Open_Result output uint8 size=1; Motor_Num input uint8 size=1; Encode_Pos output int32 size=1; PWMOUT output uint16 size=1; Temp_Down_Limit local uint32; Flag_Temp_Down output uint8; QDQ_BJ output uint8; In_State local uint8; PC1 data_store_memory double; PC2 data_store_memory double; QDQ_XH output boolean =1; QDQ_HY output boolean =1; Flag_Up_limit output uint8; Flag_Down_limit output uint8; Flag_Enc_Error output uint8; Flag_Motor_Error output uint8; Down_Limit input uint8; Encode_Sp input int32; Up_Limit input uint8; DCZD output boolean; Enc_i local uint32; can1_i local uint16; Flag_GXDY_Error output uint8; JD_In input int32; JD_Vary local uint32; GXDY_State input boolean; GXDY_IT_In input uint8; Flag_GXDY_IT output uint8; GXDY_i local uint16; KG_En data_store_memory double; KG_JD data_store_memory double; KG_YJ data_store_memory double; SGWY_In input int32 size=1; YJ_In input int32 size=1; JD_Error output int32; JD_Out output int32; SGWY_Out output int32; Cur_GZ_Limit local uint16; Flag_GZ_Cur output uint8; Flag_Up_GZ_limit output uint8; Flag_Down_GZ_limit output uint8; YJ_XHZY_HC data_store_memory double; YJ_XHZY data_store_memory double; JD_HYDG_HC data_store_memory double; JD_HYDG data_store_memory double; JD_XHHY_HC data_store_memory double; JD_XHHY data_store_memory double; JD_XHZY data_store_memory double; JD_XHZY_HC data_store_memory double; Alarm_Cunt output uint8; KG_clc data_store_memory double; KG data_store_memory double; chu_jd data_store_memory double; Encode_Pos_kj input int32 size=1; Encode_sxwPos_Motor input int32; Showing_Angle input double; Showing_T input double; Test_Mode input double; Working_Mode input double; Angle local double; Encode_Pos_Zero_Average input double; Angle_Calculation local double; Encode_Pos0 local double
  function y=Init_Result_Check(In1,In2,In3):
    | function y=Init_Result_Check(In1,In2,In3)
    |  if((In1==1)&&(In2==1)&&(In3==1))
    |      y=uint8(1);
    |  else
    |       y=uint8(0);
    |  end
